simulink model "Demo_TA2_cs"  (Simulink 7.6)
settings: Solver=FixedStepDiscrete  SolverMode=SingleTasking  StartTime=0.0  StopTime=5  FixedStep=1/60  RelTol=1e-3
model workspace (MAT data in the model file):
  mbox_table.block_array(1).src = 'built-in/Subsystem'
  mbox_table.block_array(1).dest = 'Demo_TA2_cs/BMW_X5_1'
  mbox_table.block_array(1).mode = 0
  mbox_table.block_array(2).src = 'simulink/Sinks/Out1'
  mbox_table.block_array(2).dest = 'Demo_TA2_cs/BMW_X5_1/STATE_BMW_X5_1'
  mbox_table.block_array(2).mode = 0
  mbox_table.block_array(3).src = 'PreScanSimulinkLibrary/State'
  mbox_table.block_array(3).dest = 'Demo_TA2_cs/STATE_BMW_X5_1'
  mbox_table.block_array(3).mode = 0
  mbox_table.block_array(4).src = 'PreScanSimulinkLibrary/Trajectories'
  mbox_table.block_array(4).dest = 'Demo_TA2_cs/BMW_X5_1/Trajectories'
  mbox_table.block_array(4).mode = 0
  mbox_table.block_array(5).src = 'simulink/Signal Routing/Multiport Switch'
  mbox_table.block_array(5).dest = 'Demo_TA2_cs/BMW_X5_1/Trajectories/Switch'
  mbox_table.block_array(5).mode = 0
  mbox_table.block_array(6).src = 'simulink/Sources/Constant'
  mbox_table.block_array(6).dest = 'Demo_TA2_cs/BMW_X5_1/Trajectories/Trajectory_1_Offset'
  mbox_table.block_array(6).mode = 0
  mbox_table.block_array(7).src = 'PreScanSimulinkLibrary/Trajectory'
  mbox_table.block_array(7).dest = 'Demo_TA2_cs/BMW_X5_1/Trajectories/Trajectory_1'
  mbox_table.block_array(7).mode = 0
  mbox_table.block_array(8).src = 'PreScanSimulinkLibrary/Traj2State'
  mbox_table.block_array(8).dest = 'Demo_TA2_cs/BMW_X5_1/Trajectories/Traj2State1'
  mbox_table.block_array(8).mode = 0
  mbox_table.block_array(9).src = 'simulink/Sources/Constant'
  mbox_table.block_array(9).dest = 'Demo_TA2_cs/BMW_X5_1/Trajectories/Trajectory_2_Offset'
  mbox_table.block_array(9).mode = 0
  mbox_table.block_array(10).src = 'PreScanSimulinkLibrary/Trajectory'
  mbox_table.block_array(10).dest = 'Demo_TA2_cs/BMW_X5_1/Trajectories/Trajectory_2'
  mbox_table.block_array(10).mode = 0
  mbox_table.block_array(11).src = 'PreScanSimulinkLibrary/Traj2State'
  mbox_table.block_array(11).dest = 'Demo_TA2_cs/BMW_X5_1/Trajectories/Traj2State2'
  mbox_table.block_array(11).mode = 0
  mbox_table.block_array(12).src = 'simulink/Sinks/Out1'
  mbox_table.block_array(12).dest = 'Demo_TA2_cs/BMW_X5_1/Trajectories/State'
  mbox_table.block_array(12).mode = 0
  mbox_table.block_array(13).src = 'simulink/Sources/Constant'
  mbox_table.block_array(13).dest = 'Demo_TA2_cs/BMW_X5_1/Trajectories/SelectTraj'
  mbox_table.block_array(13).mode = 0
  mbox_table.block_array(14).src = 'PreScanSimulinkLibrary/SELF'
  mbox_table.block_array(14).dest = 'Demo_TA2_cs/SELF_BMW_X5_1'
  mbox_table.block_array(14).mode = 0
  mbox_table.block_array(15).src = 'simulink/Sources/In1'
  mbox_table.block_array(15).dest = 'Demo_TA2_cs/BMW_X5_1/SELF_BMW_X5_1'
  mbox_table.block_array(15).mode = 0
  mbox_table.block_array(16).src = 'PreScanSimulinkLibrary/DemuxSELF'
  mbox_table.block_array(16).dest = 'Demo_TA2_cs/BMW_X5_1/SELF_Demux'
  mbox_table.block_array(16).mode = 0
  mbox_table.block_array(17).src = 'built-in/S-Function'
  mbox_table.block_array(17).dest = 'Demo_TA2_cs/TIS_1'
  mbox_table.block_array(17).mode = 0
  mbox_table.block_array(18).src = 'simulink/Sources/In1'
  mbox_table.block_array(18).dest = 'Demo_TA2_cs/BMW_X5_1/TIS_1'
  mbox_table.block_array(18).mode = 0
  mbox_table.block_array(19).src = 'PreScanSimulinkLibrary/DemuxTIS_Standard'
  mbox_table.block_array(19).dest = 'Demo_TA2_cs/BMW_X5_1/TIS_1_Standard_Demux'
  mbox_table.block_array(19).mode = 0
  mbox_table.block_array(20).src = 'built-in/Subsystem'
  mbox_table.block_array(20).dest = 'Demo_TA2_cs/Box_1'
  mbox_table.block_array(20).mode = 0
  mbox_table.block_array(21).src = 'simulink/Sinks/Out1'
  mbox_table.block_array(21).dest = 'Demo_TA2_cs/Box_1/STATE_Box_1'
  mbox_table.block_array(21).mode = 0
  mbox_table.block_array(22).src = 'PreScanSimulinkLibrary/State'
  mbox_table.block_array(22).dest = 'Demo_TA2_cs/STATE_Box_1'
  mbox_table.block_array(22).mode = 0
  mbox_table.block_array(23).src = 'PreScanSimulinkLibrary/SELF'
  mbox_table.block_array(23).dest = 'Demo_TA2_cs/SELF_Box_1'
  mbox_table.block_array(23).mode = 0
  mbox_table.block_array(24).src = 'simulink/Sources/In1'
  mbox_table.block_array(24).dest = 'Demo_TA2_cs/Box_1/SELF_Box_1'
  mbox_table.block_array(24).mode = 0
  mbox_table.block_array(25).src = 'PreScanSimulinkLibrary/DemuxSELF'
  mbox_table.block_array(25).dest = 'Demo_TA2_cs/Box_1/SELF_Demux'
  mbox_table.block_array(25).mode = 0
  mbox_table.block_array(26).src = 'built-in/Subsystem'
  mbox_table.block_array(26).dest = 'Demo_TA2_cs/Box_1/Dynamics_Empty'
  mbox_table.block_array(26).mode = 0
  mbox_table.block_array(27).src = 'PreScanSimulinkLibrary/MuxState'
  mbox_table.block_array(27).dest = 'Demo_TA2_cs/Box_1/Dynamics_Empty/MuxState'
  mbox_table.block_array(27).mode = 0
  mbox_table.block_array(28).src = 'simulink/Sinks/Out1'
  mbox_table.block_array(28).dest = 'Demo_TA2_cs/Box_1/Dynamics_Empty/State'
  mbox_table.block_array(28).mode = 0
  mbox_table.block_array(29).src = 'built-in/Note'
  mbox_table.block_array(29).dest = 'Demo_TA2_cs/Box_1/Dynamics_Empty/For state mode ''Dynamic'' positions
    | are not taken into account, as they
    | are computed by integrating velocity.
    | Click annotation for Help.'
  mbox_table.block_array(29).mode = 0
  mbox_table.block_array(30).src = 'SimCoreLibrary/SimCoreConfiguration'
  mbox_table.block_array(30).dest = 'Demo_TA2_cs/SimCoreConfiguration'
  mbox_table.block_array(30).mode = 0
  mbox_table.block_array(31).src = 'SimCoreLibrary/Actuators'
  mbox_table.block_array(31).dest = 'Demo_TA2_cs/Actuators'
  mbox_table.block_array(31).mode = 0
  mbox_table.block_array(32).src = 'SimCoreLibrary/SetActuators'
  mbox_table.block_array(32).dest = 'Demo_TA2_cs/SetActuators'
  mbox_table.block_array(32).mode = 0
  mbox_table.block_array(33).src = 'SimCoreLibrary/GetSensors'
  mbox_table.block_array(33).dest = 'Demo_TA2_cs/GetSensors'
  mbox_table.block_array(33).mode = 0
  mbox_table.block_array(34).src = 'SimCoreLibrary/SimCoreInfo'
  mbox_table.block_array(34).dest = 'Demo_TA2_cs/SimCoreInfo'
  mbox_table.block_array(34).mode = 0
  mbox_table.block_array(35).src = 'PreScanSimulinkLibrary/Regenerate'
  mbox_table.block_array(35).dest = 'Demo_TA2_cs/Regenerate'
  mbox_table.block_array(35).mode = 0
  mbox_table.block_array(36).src = 'PreScanSimulinkLibrary/Record for Replay  '
  mbox_table.block_array(36).dest = 'Demo_TA2_cs/Record for Replay  '
  mbox_table.block_array(36).mode = 0
  mbox_table.block_array(37).src = 'PreScanSimulinkLibrary/Open Useful Blocks'
  mbox_table.block_array(37).dest = 'Demo_TA2_cs/Open Useful Blocks'
  mbox_table.block_array(37).mode = 0
  mbox_table.block_array(38).src = 'PreScanSimulinkLibrary/PreScan Options   '
  mbox_table.block_array(38).dest = 'Demo_TA2_cs/PreScan Options   '
  mbox_table.block_array(38).mode = 0
  mbox_table.block_array(39).src = 'built-in/Note'
  mbox_table.block_array(39).dest = 'Demo_TA2_cs/Version:                  '
  mbox_table.block_array(39).mode = 0
  mbox_table.block_array(40).src = 'built-in/Note'
  mbox_table.block_array(40).dest = 'Demo_TA2_cs/7.4.0'
  mbox_table.block_array(40).mode = 0
  mbox_table.block_array(41).src = 'built-in/Note'
  mbox_table.block_array(41).dest = 'Demo_TA2_cs/Author(s):                '
  mbox_table.block_array(41).mode = 0
  mbox_table.block_array(42).src = 'built-in/Note'
  mbox_table.block_array(42).dest = 'Demo_TA2_cs/D. Terra'
  mbox_table.block_array(42).mode = 0
  mbox_table.block_array(43).src = 'built-in/Note'
  mbox_table.block_array(43).dest = 'Demo_TA2_cs/Descriptive text:      '
  mbox_table.block_array(43).mode = 0
  mbox_table.block_array(44).src = 'built-in/Note'
  mbox_table.block_array(44).dest = 'Demo_TA2_cs/This experiment illustrates the
    | possibilities for Test Automation
    | that requires the PreScan
    | Experiment Editor to rebuild the
    | scenario.'
  mbox_table.block_array(44).mode = 0
  mbox_table.block_array(45).src = 'built-in/Note'
  mbox_table.block_array(45).dest = 'Demo_TA2_cs/ID
    | 
    | 4
    | 9'
  mbox_table.block_array(45).mode = 0
  mbox_table.block_array(46).src = 'built-in/Note'
  mbox_table.block_array(46).dest = 'Demo_TA2_cs/OBU-Beacon ID
    | 
    | 
    | '
  mbox_table.block_array(46).mode = 0
  mbox_table.block_array(47).src = 'built-in/Note'
  mbox_table.block_array(47).dest = 'Demo_TA2_cs/TypeID
    | 
    | 1
    | 5'
  mbox_table.block_array(47).mode = 0
  mbox_table.block_array(48).src = 'built-in/Note'
  mbox_table.block_array(48).dest = 'Demo_TA2_cs/TypeTag
    | 
    | Car
    | Cal element'
  mbox_table.block_array(48).mode = 0
  mbox_table.block_array(49).src = 'built-in/Note'
  mbox_table.block_array(49).dest = 'Demo_TA2_cs/SD
    | 
    | Y
    | Y'
  mbox_table.block_array(49).mode = 0
  mbox_table.block_array(50).src = 'built-in/Note'
  mbox_table.block_array(50).dest = 'Demo_TA2_cs/CD
    | 
    | N
    | N'
  mbox_table.block_array(50).mode = 0
  mbox_table.block_array(51).src = 'built-in/Note'
  mbox_table.block_array(51).dest = 'Demo_TA2_cs/Name
    | 
    | BMW_X5_1
    | Box_1'
  mbox_table.block_array(51).mode = 0
  mbox_table.block_array(52).src = 'built-in/Note'
  mbox_table.block_array(52).dest = 'Demo_TA2_cs/Num ID       OBU-Beacon ID     Type ID      Type Tag             SD        CD             Name                          '
  mbox_table.block_array(52).mode = 0
  mbox_table.block_array(53).src = 'built-in/Terminator'
  mbox_table.block_array(53).dest = 'Demo_TA2_cs/BMW_X5_1/Terminator_1'
  mbox_table.block_array(53).mode = 1
  mbox_table.block_array(54).src = 'built-in/Terminator'
  mbox_table.block_array(54).dest = 'Demo_TA2_cs/BMW_X5_1/Terminator_2'
  mbox_table.block_array(54).mode = 1
  mbox_table.block_array(55).src = 'built-in/Terminator'
  mbox_table.block_array(55).dest = 'Demo_TA2_cs/BMW_X5_1/Terminator_3'
  mbox_table.block_array(55).mode = 1
  mbox_table.block_array(56).src = 'built-in/Terminator'
  mbox_table.block_array(56).dest = 'Demo_TA2_cs/BMW_X5_1/Terminator_4'
  mbox_table.block_array(56).mode = 1
  mbox_table.block_array(57).src = 'built-in/Terminator'
  mbox_table.block_array(57).dest = 'Demo_TA2_cs/BMW_X5_1/Terminator_5'
  mbox_table.block_array(57).mode = 1
  mbox_table.block_array(58).src = 'built-in/Terminator'
  mbox_table.block_array(58).dest = 'Demo_TA2_cs/BMW_X5_1/Terminator_6'
  mbox_table.block_array(58).mode = 1
  mbox_table.block_array(59).src = 'built-in/Terminator'
  mbox_table.block_array(59).dest = 'Demo_TA2_cs/BMW_X5_1/Terminator_7'
  mbox_table.block_array(59).mode = 1
  mbox_table.block_array(60).src = 'built-in/Terminator'
  mbox_table.block_array(60).dest = 'Demo_TA2_cs/BMW_X5_1/Terminator_8'
  mbox_table.block_array(60).mode = 1
  mbox_table.block_array(61).src = 'built-in/Terminator'
  mbox_table.block_array(61).dest = 'Demo_TA2_cs/BMW_X5_1/Terminator_9'
  mbox_table.block_array(61).mode = 1
  mbox_table.block_array(62).src = 'built-in/Terminator'
  mbox_table.block_array(62).dest = 'Demo_TA2_cs/BMW_X5_1/Terminator_10'
  mbox_table.block_array(62).mode = 1
  mbox_table.block_array(63).src = 'built-in/Terminator'
  mbox_table.block_array(63).dest = 'Demo_TA2_cs/BMW_X5_1/Terminator_11'
  mbox_table.block_array(63).mode = 1
  mbox_table.block_array(64).src = 'built-in/Terminator'
  mbox_table.block_array(64).dest = 'Demo_TA2_cs/BMW_X5_1/Terminator_12'
  mbox_table.block_array(64).mode = 1
  mbox_table.block_array(65).src = 'built-in/Terminator'
  mbox_table.block_array(65).dest = 'Demo_TA2_cs/BMW_X5_1/Terminator_13'
  mbox_table.block_array(65).mode = 1
  mbox_table.block_array(66).src = 'built-in/Terminator'
  mbox_table.block_array(66).dest = 'Demo_TA2_cs/BMW_X5_1/Terminator_14'
  mbox_table.block_array(66).mode = 1
  mbox_table.block_array(67).src = 'built-in/Terminator'
  mbox_table.block_array(67).dest = 'Demo_TA2_cs/BMW_X5_1/Terminator_15'
  mbox_table.block_array(67).mode = 1
  mbox_table.block_array(68).src = 'built-in/Terminator'
  mbox_table.block_array(68).dest = 'Demo_TA2_cs/BMW_X5_1/Terminator_16'
  mbox_table.block_array(68).mode = 1
  mbox_table.block_index : java.util.Hashtable (value not decoded)
  mbox_table.line_array(1).sys = 'Demo_TA2_cs'
  mbox_table.line_array(1).line_id = 'L1'
  mbox_table.line_array(1).iport = 'STATE_BMW_X5_1/1'
  mbox_table.line_array(1).oport = 'BMW_X5_1/1'
  mbox_table.line_array(1).mode = 0
  mbox_table.line_array(2).sys = 'Demo_TA2_cs/BMW_X5_1/Trajectories'
  mbox_table.line_array(2).line_id = 'L2'
  mbox_table.line_array(2).iport = 'Traj2State1/1'
  mbox_table.line_array(2).oport = 'Trajectory_1/1'
  mbox_table.line_array(2).mode = 0
  mbox_table.line_array(3).sys = 'Demo_TA2_cs/BMW_X5_1/Trajectories'
  mbox_table.line_array(3).line_id = 'L3'
  mbox_table.line_array(3).iport = 'Traj2State1/2'
  mbox_table.line_array(3).oport = 'Trajectory_1_Offset/1'
  mbox_table.line_array(3).mode = 0
  mbox_table.line_array(4).sys = 'Demo_TA2_cs/BMW_X5_1/Trajectories'
  mbox_table.line_array(4).line_id = 'L4'
  mbox_table.line_array(4).iport = 'Switch/2'
  mbox_table.line_array(4).oport = 'Traj2State1/1'
  mbox_table.line_array(4).mode = 0
  mbox_table.line_array(5).sys = 'Demo_TA2_cs/BMW_X5_1/Trajectories'
  mbox_table.line_array(5).line_id = 'L5'
  mbox_table.line_array(5).iport = 'Traj2State2/1'
  mbox_table.line_array(5).oport = 'Trajectory_2/1'
  mbox_table.line_array(5).mode = 0
  mbox_table.line_array(6).sys = 'Demo_TA2_cs/BMW_X5_1/Trajectories'
  mbox_table.line_array(6).line_id = 'L6'
  mbox_table.line_array(6).iport = 'Traj2State2/2'
  mbox_table.line_array(6).oport = 'Trajectory_2_Offset/1'
  mbox_table.line_array(6).mode = 0
  mbox_table.line_array(7).sys = 'Demo_TA2_cs/BMW_X5_1/Trajectories'
  mbox_table.line_array(7).line_id = 'L7'
  mbox_table.line_array(7).iport = 'Switch/3'
  mbox_table.line_array(7).oport = 'Traj2State2/1'
  mbox_table.line_array(7).mode = 0
  mbox_table.line_array(8).sys = 'Demo_TA2_cs/BMW_X5_1/Trajectories'
  mbox_table.line_array(8).line_id = 'L8'
  mbox_table.line_array(8).iport = 'Switch/1'
  mbox_table.line_array(8).oport = 'SelectTraj/1'
  mbox_table.line_array(8).mode = 0
  mbox_table.line_array(9).sys = 'Demo_TA2_cs/BMW_X5_1/Trajectories'
  mbox_table.line_array(9).line_id = 'L9'
  mbox_table.line_array(9).iport = 'State/1'
  mbox_table.line_array(9).oport = 'Switch/1'
  mbox_table.line_array(9).mode = 0
  mbox_table.line_array(10).sys = 'Demo_TA2_cs'
  mbox_table.line_array(10).line_id = 'L10'
  mbox_table.line_array(10).iport = 'BMW_X5_1/1'
  mbox_table.line_array(10).oport = 'SELF_BMW_X5_1/1'
  mbox_table.line_array(10).mode = 0
  mbox_table.line_array(11).sys = 'Demo_TA2_cs/BMW_X5_1'
  mbox_table.line_array(11).line_id = 'L11'
  mbox_table.line_array(11).iport = 'SELF_Demux/1'
  mbox_table.line_array(11).oport = 'SELF_BMW_X5_1/1'
  mbox_table.line_array(11).mode = 0
  mbox_table.line_array(12).sys = 'Demo_TA2_cs'
  mbox_table.line_array(12).line_id = 'L12'
  mbox_table.line_array(12).iport = 'BMW_X5_1/2'
  mbox_table.line_array(12).oport = 'TIS_1/1'
  mbox_table.line_array(12).mode = 0
  mbox_table.line_array(13).sys = 'Demo_TA2_cs/BMW_X5_1'
  mbox_table.line_array(13).line_id = 'L13'
  mbox_table.line_array(13).iport = 'TIS_1_Standard_Demux/1'
  mbox_table.line_array(13).oport = 'TIS_1/1'
  mbox_table.line_array(13).mode = 0
  mbox_table.line_array(14).sys = 'Demo_TA2_cs/BMW_X5_1'
  mbox_table.line_array(14).line_id = 'L14'
  mbox_table.line_array(14).iport = 'STATE_BMW_X5_1/1'
  mbox_table.line_array(14).oport = 'Trajectories/1'
  mbox_table.line_array(14).mode = 0
  mbox_table.line_array(15).sys = 'Demo_TA2_cs'
  mbox_table.line_array(15).line_id = 'L15'
  mbox_table.line_array(15).iport = 'STATE_Box_1/1'
  mbox_table.line_array(15).oport = 'Box_1/1'
  mbox_table.line_array(15).mode = 0
  mbox_table.line_array(16).sys = 'Demo_TA2_cs'
  mbox_table.line_array(16).line_id = 'L16'
  mbox_table.line_array(16).iport = 'Box_1/1'
  mbox_table.line_array(16).oport = 'SELF_Box_1/1'
  mbox_table.line_array(16).mode = 0
  mbox_table.line_array(17).sys = 'Demo_TA2_cs/Box_1'
  mbox_table.line_array(17).line_id = 'L17'
  mbox_table.line_array(17).iport = 'SELF_Demux/1'
  mbox_table.line_array(17).oport = 'SELF_Box_1/1'
  mbox_table.line_array(17).mode = 0
  mbox_table.line_array(18).sys = 'Demo_TA2_cs/Box_1/Dynamics_Empty'
  mbox_table.line_array(18).line_id = 'L18'
  mbox_table.line_array(18).iport = 'State/1'
  mbox_table.line_array(18).oport = 'MuxState/1'
  mbox_table.line_array(18).mode = 0
  mbox_table.line_array(19).sys = 'Demo_TA2_cs/Box_1'
  mbox_table.line_array(19).line_id = 'L19'
  mbox_table.line_array(19).iport = 'STATE_Box_1/1'
  mbox_table.line_array(19).oport = 'Dynamics_Empty/1'
  mbox_table.line_array(19).mode = 0
  mbox_table.line_array(20).sys = 'Demo_TA2_cs/BMW_X5_1'
  mbox_table.line_array(20).line_id = 'l1'
  mbox_table.line_array(20).iport = 'Terminator_1/1'
  mbox_table.line_array(20).oport = 'SELF_Demux/1'
  mbox_table.line_array(20).mode = 1
  mbox_table.line_array(21).sys = 'Demo_TA2_cs/BMW_X5_1'
  mbox_table.line_array(21).line_id = 'l2'
  mbox_table.line_array(21).iport = 'Terminator_2/1'
  mbox_table.line_array(21).oport = 'SELF_Demux/2'
  mbox_table.line_array(21).mode = 1
  mbox_table.line_array(22).sys = 'Demo_TA2_cs/BMW_X5_1'
  mbox_table.line_array(22).line_id = 'l3'
  mbox_table.line_array(22).iport = 'Terminator_3/1'
  mbox_table.line_array(22).oport = 'SELF_Demux/3'
  mbox_table.line_array(22).mode = 1
  mbox_table.line_array(23).sys = 'Demo_TA2_cs/BMW_X5_1'
  mbox_table.line_array(23).line_id = 'l4'
  mbox_table.line_array(23).iport = 'Terminator_4/1'
  mbox_table.line_array(23).oport = 'SELF_Demux/4'
  mbox_table.line_array(23).mode = 1
  mbox_table.line_array(24).sys = 'Demo_TA2_cs/BMW_X5_1'
  mbox_table.line_array(24).line_id = 'l5'
  mbox_table.line_array(24).iport = 'Terminator_5/1'
  mbox_table.line_array(24).oport = 'SELF_Demux/5'
  mbox_table.line_array(24).mode = 1
  mbox_table.line_array(25).sys = 'Demo_TA2_cs/BMW_X5_1'
  mbox_table.line_array(25).line_id = 'l6'
  mbox_table.line_array(25).iport = 'Terminator_6/1'
  mbox_table.line_array(25).oport = 'SELF_Demux/6'
  mbox_table.line_array(25).mode = 1
  mbox_table.line_array(26).sys = 'Demo_TA2_cs/BMW_X5_1'
  mbox_table.line_array(26).line_id = 'l7'
  mbox_table.line_array(26).iport = 'Terminator_7/1'
  mbox_table.line_array(26).oport = 'SELF_Demux/7'
  mbox_table.line_array(26).mode = 1
  mbox_table.line_array(27).sys = 'Demo_TA2_cs/BMW_X5_1'
  mbox_table.line_array(27).line_id = 'l8'
  mbox_table.line_array(27).iport = 'Terminator_8/1'
  mbox_table.line_array(27).oport = 'SELF_Demux/8'
  mbox_table.line_array(27).mode = 1
  mbox_table.line_array(28).sys = 'Demo_TA2_cs/BMW_X5_1'
  mbox_table.line_array(28).line_id = 'l9'
  mbox_table.line_array(28).iport = 'Terminator_9/1'
  mbox_table.line_array(28).oport = 'SELF_Demux/9'
  mbox_table.line_array(28).mode = 1
  mbox_table.line_array(29).sys = 'Demo_TA2_cs/BMW_X5_1'
  mbox_table.line_array(29).line_id = 'l10'
  mbox_table.line_array(29).iport = 'Terminator_10/1'
  mbox_table.line_array(29).oport = 'SELF_Demux/10'
  mbox_table.line_array(29).mode = 1
  mbox_table.line_array(30).sys = 'Demo_TA2_cs/BMW_X5_1'
  mbox_table.line_array(30).line_id = 'l11'
  mbox_table.line_array(30).iport = 'Terminator_11/1'
  mbox_table.line_array(30).oport = 'SELF_Demux/11'
  mbox_table.line_array(30).mode = 1
  mbox_table.line_array(31).sys = 'Demo_TA2_cs/BMW_X5_1'
  mbox_table.line_array(31).line_id = 'l12'
  mbox_table.line_array(31).iport = 'Terminator_12/1'
  mbox_table.line_array(31).oport = 'SELF_Demux/12'
  mbox_table.line_array(31).mode = 1
  mbox_table.line_array(32).sys = 'Demo_TA2_cs/BMW_X5_1'
  mbox_table.line_array(32).line_id = 'l13'
  mbox_table.line_array(32).iport = 'Terminator_13/1'
  mbox_table.line_array(32).oport = 'TIS_1_Standard_Demux/3'
  mbox_table.line_array(32).mode = 1
  mbox_table.line_array(33).sys = 'Demo_TA2_cs/BMW_X5_1'
  mbox_table.line_array(33).line_id = 'l14'
  mbox_table.line_array(33).iport = 'Terminator_14/1'
  mbox_table.line_array(33).oport = 'TIS_1_Standard_Demux/4'
  mbox_table.line_array(33).mode = 1
  mbox_table.line_array(34).sys = 'Demo_TA2_cs/BMW_X5_1'
  mbox_table.line_array(34).line_id = 'l15'
  mbox_table.line_array(34).iport = 'Terminator_15/1'
  mbox_table.line_array(34).oport = 'TIS_1_Standard_Demux/5'
  mbox_table.line_array(34).mode = 1
  mbox_table.line_array(35).sys = 'Demo_TA2_cs/BMW_X5_1'
  mbox_table.line_array(35).line_id = 'l16'
  mbox_table.line_array(35).iport = 'Terminator_16/1'
  mbox_table.line_array(35).oport = 'TIS_1_Standard_Demux/6'
  mbox_table.line_array(35).mode = 1
  mbox_table.line_index : java.util.Hashtable (value not decoded)
  mbox_table.next_linenr = 20
  mbox_table.next_termlinenr = 17
  model_closed = 0
  sim_status = 0
PreLoadFcn:
  | check_NUTS_defined;
  | 
  | assignin('base',['model_closed_' bdroot],false);
InitFcn:
  | PreScanExperimentInitFcn(bdroot)
StopFcn:
  | PreScanExperimentStopFcn(bdroot)
undefined symbols (not defined in the file or in its folder): DiscIntNeverNeededParam
libraries: PreScanSimulinkLibrary x9, PreScanUsefulBlocks x3
(part 1 of 2)
CloseFcn:
  | evalin('base',['clear model_closed_' bdroot]);
settings Model: Creator=PRESCAN  LastModifiedBy=buildbot
settings OptimizationCC: InitFltsAndDblsToZero=on
settings DebuggingCC: SaveWithParameterizedLinksMsg=none  SignalResolutionControl=TryResolveAllWithWarning  MultiTaskDSMMsg=warning  MultiTaskCondExecSysMsg=none
settings RTWCC: IncludeERTFirstTime=on
settings GRTTargetCC: TargetFcnLib=ansi_tfl_tmw.mat

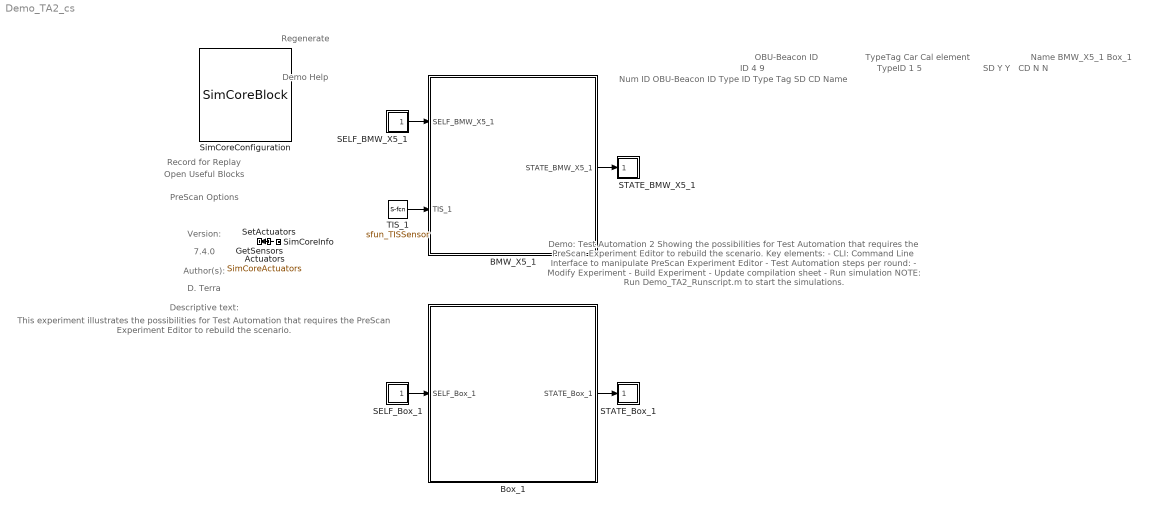
== system Demo_TA2_cs ==
  note: Demo: Test Automation 2
      | Showing the possibilities for Test Automation that requires the PreScan
      | Experiment Editor to rebuild the scenario.
      |
      | Key elements:
      | - CLI: Command Line Interface to manipulate PreScan Experiment Editor
      | - Test Automation steps per round:
      |     - Modify Experiment
      |     - Build Experiment
      |     - Update compilation sheet
      |     - Run simulation
      |
      | NOTE:
      | Run Demo_TA2_Runscript.m to start the simulations.
  note: Demo Help
  note: Regenerate
  note: Record for Replay
  note: Open Useful Blocks
  note: PreScan Options
  note: Version:
  note: 7.4.0
  note: Author(s):
  note: D. Terra
  note: Descriptive text:
  note: This experiment illustrates the
      | possibilities for Test Automation
      | that requires the PreScan
      | Experiment Editor to rebuild the
      | scenario.
  note: ID
      |
      | 4
      | 9
  note: OBU-Beacon ID
  note: TypeID
      |
      | 1
      | 5
  note: TypeTag
      |
      | Car
      | Cal element
  note: SD
      |
      | Y
      | Y
  note: CD
      |
      | N
      | N
  note: Name
      |
      | BMW_X5_1
      | Box_1
  note: Num ID OBU-Beacon ID Type ID Type Tag SD CD Name
  Actuators : DataStoreMemory  Tag=Actuators  DataStoreName=SimCoreActuators  InitialValue=zeros(30,1)
      settings: DeleteFcn=PreScanBlockDeleteFcn;
  BMW_X5_1 : Subsystem  Tag=WorldObjectSubSystem  InitFcn=UniqueId = '33';
      mask Display: image(imread('BMW_X5.jpg'));color('white');text(0,0,' ID=4\n')
  Box_1 : Subsystem  Tag=WorldObjectSubSystem  InitFcn=UniqueId = '41';
      mask Display: image(imread('Box.jpg'));color('white');text(0,0,' ID=9\n')
  GetSensors : Subsystem  Tag=GetSensors  Priority=2  mask(PreScan Simulation Core Block){NrOfSensors=16, TimeStep=1/60}
      mask prompts: NrOfSensors "Number of sensor values"; TimeStep "Timestep [s]"
      mask help:
      | Please do not remove this block from the PreScan compilation sheet,
      | as it contains essential configuration parameters for a PreScan simulation.
      settings: DeleteFcn=PreScanBlockDeleteFcn;
  SELF_BMW_X5_1 : Subsystem  Tag=SELF  Priority=3  mask(PreScan Source Block: SELF){PortName=SELF_BMW_X5_1, PortIndex=0, PortWidth=8, TimeStep=1/60}
      mask prompts: PortName "Auto-Assigned: Port Name [-]"; PortIndex "Auto-Assigned: Port Index [-]"; PortWidth "Auto-Assigned: Port Dimensions"; TimeStep "Auto-Assigned: Upload Period [s]"
      mask help:
      | The SELF port shows (state) information of the actor itself. The outputs are position in the experiment's axis system and the GPS coordinates, and the object's absolute velocity and compass heading.
      |
      | For more information, please click Help.
      settings: DeleteFcn=PreScanBlockDeleteFcn;
      mask Help: eval('openHelp(462)')
      mask Display: image(imread('GPS.png'))
  SELF_Box_1 : Subsystem  Tag=SELF  Priority=3  mask(PreScan Source Block: SELF){PortName=SELF_Box_1, PortIndex=8, PortWidth=8, TimeStep=1/60}
      mask prompts: PortName "Auto-Assigned: Port Name [-]"; PortIndex "Auto-Assigned: Port Index [-]"; PortWidth "Auto-Assigned: Port Dimensions"; TimeStep "Auto-Assigned: Upload Period [s]"
      mask help:
      | The SELF port shows (state) information of the actor itself. The outputs are position in the experiment's axis system and the GPS coordinates, and the object's absolute velocity and compass heading.
      |
      | For more information, please click Help.
      settings: DeleteFcn=PreScanBlockDeleteFcn;
      mask Help: eval('openHelp(462)')
      mask Display: image(imread('GPS.png'))
  STATE_BMW_X5_1 : Subsystem  Tag=State  Priority=0  mask(PreScan Sink Block: State){x0=0, y0=-1.75, z0=0.68999999761581421, Roll0=0, Pitch0=0, Yaw0=0, TimeStep=1/60}
      mask prompts: x0 "Ini x-position VEHICLE wrt GLOBAL axis system [m]"; y0 "Ini y-position VEHICLE wrt GLOBAL axis system [m]"; z0 "Ini z-position VEHICLE wrt GLOBAL axis system [m]"; Roll0 "Ini roll-angle BODY wrt VEHICLE axis system [deg]"; Pitch0 "Ini pitch-angle BODY wrt VEHICLE axis system [deg]"; Yaw0 "Ini yaw-angle VEHICLE wrt GLOBAL axis system [deg]"; TimeStep "Time Step [s]"
      mask help:
      | The Actor State contains a vector signal of size (9x1), containing the following signals:
      |
      | -  Position                  (x,y,z)                                     [m]
      | -  Velocity                  (vx,vy,vz)                               [m/s]
      | -  Angles                    (Roll, Pitch, Yaw)                   [rad]
      |
      | The Actor state is defined in the global axis system.
      | The state is superponed on the Initial position defined in the GUI.
      |
      | For more information, please click Help.
      settings: DeleteFcn=PreScanBlockDeleteFcn;
      mask Help: eval('openHelp(222)')
      mask Display: image(imread('State.png'))
  STATE_Box_1 : Subsystem  Tag=State  Priority=0  mask(PreScan Sink Block: State){x0=38, y0=0, z0=0, Roll0=0, Pitch0=0, Yaw0=0, TimeStep=1/60}
      mask prompts: x0 "Ini x-position VEHICLE wrt GLOBAL axis system [m]"; y0 "Ini y-position VEHICLE wrt GLOBAL axis system [m]"; z0 "Ini z-position VEHICLE wrt GLOBAL axis system [m]"; Roll0 "Ini roll-angle BODY wrt VEHICLE axis system [deg]"; Pitch0 "Ini pitch-angle BODY wrt VEHICLE axis system [deg]"; Yaw0 "Ini yaw-angle VEHICLE wrt GLOBAL axis system [deg]"; TimeStep "Time Step [s]"
      mask help:
      | The Actor State contains a vector signal of size (9x1), containing the following signals:
      |
      | -  Position                  (x,y,z)                                     [m]
      | -  Velocity                  (vx,vy,vz)                               [m/s]
      | -  Angles                    (Roll, Pitch, Yaw)                   [rad]
      |
      | The Actor state is defined in the global axis system.
      | The state is superponed on the Initial position defined in the GUI.
      |
      | For more information, please click Help.
      settings: DeleteFcn=PreScanBlockDeleteFcn;
      mask Help: eval('openHelp(222)')
      mask Display: image(imread('State.png'))
  SetActuators : Subsystem  Tag=SetActuators  Priority=1  mask(PreScan Simulation Core Block){TimeStep=1/60, NrOfActuators=30}
      mask prompts: TimeStep "Timestep [s]"; NrOfActuators "Number of actuator values"
      mask help:
      | Please do not remove this block from the PreScan compilation sheet,
      | as it contains essential configuration parameters for a PreScan simulation.
      settings: DeleteFcn=PreScanBlockDeleteFcn;
  SimCoreConfiguration : M-S-Function  Tag=SimCoreConfiguration  Description=839168CDEDD100B1BE966240BE789E2F4508DB343ED6100BC12AAB51D6F7B04F  FunctionName=SimCoreBlock  Parameters=ExperimentXML PortsXML SimulationCore HostName CheckStart EnableLog RfR EnableGPUAccel ShowComputationTime  mask(PreScan Simulation Core Configurator){SimulationCore=NUTS, HostName=0, CheckStart=0, prescanversion='7.4.0', EnableLog=off, RfR=0, EnableGPUAccel=off, ShowComputationTime=off}
      mask prompts: SimulationCore "Simulation Core"; HostName "Simulation Host"; CheckStart "Show START Dialog"; prescanversion "PreScan Version"; EnableLog "Create TA Log"; RfR "Record for Replay"; EnableGPUAccel "Enable GPU Acceleration"; ShowComputationTime "Show ComputationTime Scope"
      mask help:
      | Please do not remove this block from the PreScan compilation sheet,
      | as it contains essential configuration parameter for a PreScan simulation.
      mask init:
      | model = bdroot;
      | ExperimentXML = [model(1:end-3) '.pex'];
      | PortsXML = [model '_ports.pcd'];
      settings: DeleteFcn=PreScanBlockDeleteFcn;  ModelCloseFcn=assignin('base',['model_closed_' bdroot],true);
      mask Help: eval('openHelp(812)')
      mask Display: image(imread('prescanlogo.ico'))
  SimCoreInfo : Subsystem  Tag=SimCoreInfo
  TIS_1 : S-Function  Priority=3  LoadFcn=load('PrescanScannerSensorData.mat');load('PrescanScannerSensorMessage.mat')  FunctionName=sfun_TISSensor  Parameters=timestepMask maxInputMessages maxOutputMessages sensorID detectableObjects  EnableBusSupport=off  mask{timestepMask=1/60, maxInputMessages=0, maxOutputMessages=1, sensorID=40, detectableObjects=1}
      mask prompts: timestepMask "MATLAB timestep:"; maxInputMessages "Max input messages:"; maxOutputMessages "Max output messages:"; sensorID "Sensor ID:"; detectableObjects "Max detectable objects:"
      mask help: TIS Sensor I/O
      mask Display: image(imread('TIS.png'))
  wires:
  BMW_X5_1/1(STATE_BMW_X5_1) -> STATE_BMW_X5_1/1(State)
  SELF_BMW_X5_1/1(U) -> BMW_X5_1/1(SELF_BMW_X5_1)
  TIS_1/1 -> BMW_X5_1/2(TIS_1)
  Box_1/1(STATE_Box_1) -> STATE_Box_1/1(State)
  SELF_Box_1/1(U) -> Box_1/1(SELF_Box_1)
  SetActuators/1(dummy) -> GetSensors/1(dummy)

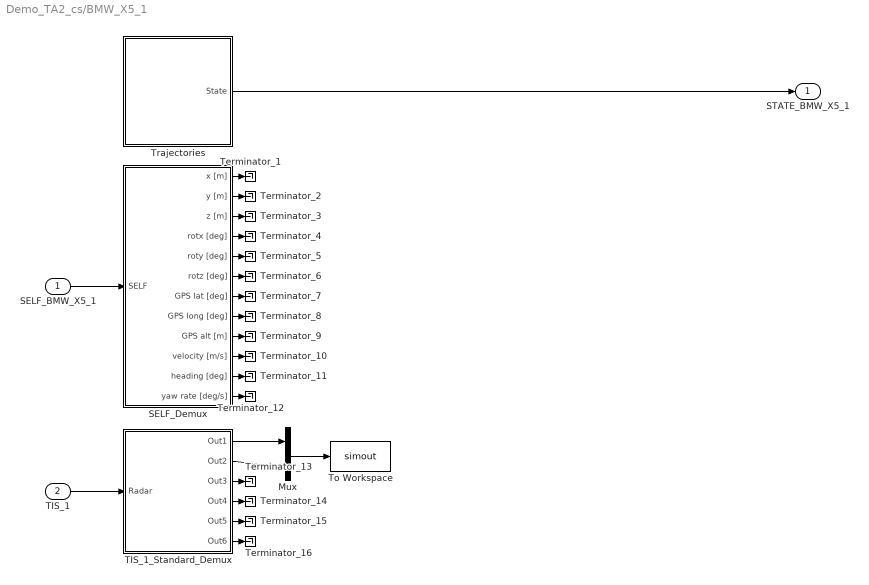
== system Demo_TA2_cs/BMW_X5_1 ==
  SELF_BMW_X5_1 : Inport  Tag=SELFInport
  TIS_1 : Inport  Tag=RadarInport  Port=2  OutDataTypeStr=Bus: PRESCAN_SCANNERSENSORMESSAGE
  Mux : Mux  Inputs=2
  SELF_Demux : Subsystem  Tag=DemuxSELF
      settings: DeleteFcn=PreScanBlockDeleteFcn;
      mask Type: PreScan Demux Block:
      mask Display:
      | port_label('output',1,'x [m]')
      | port_label('output',2,'y [m]')
      | port_label('output',3,'z [m]','texmode','on')
      | port_label('output',4,'Rotx [deg]','texmode','on')
      | port_label('output',5,'Roty [deg]','texmode','on')
      | port_label('output',6,'Rotz [deg]','texmode','on')
      | port_label('output',7,'GPS lat [deg]','texmode','on')
      | port_label('output',8,'GPS long [deg]','texmode','on')
      | port_label('output',9,'GPS alt [m]','texmode','on')
      | port_label('output',10,'Velocity [m/s]')
      | port_label('output',11,'Heading [deg]')
      | port_label('output',12,'Yaw rate [deg/s]')
  TIS_1_Standard_Demux : Subsystem  TreatAsAtomicUnit=on  mask(PreScan Demux Block: TIS){MAXMESSAGES=1}
      mask prompts: MAXMESSAGES "Number of Objects"
      mask Help: eval('openHelp(441)')
      mask Display:
      | port_label('input',1,'TIS')
      | port_label('output',1,'Beam ID [-]')
      | port_label('output',2,'Range [m]')
      | port_label('output',3,'{\theta} [deg]','texmode','on')
      | port_label('output',4,'{\phi} [deg]','texmode','on')
      | port_label('output',5,'Target ID [-]','texmode','on')
      | port_label('output',6,'TIS Data','texmode','on')
  Terminator_{1..16} (16 alike) : Terminator
  To Workspace : ToWorkspace  VariableName=simout  SampleTime=-1  SaveFormat=Array
  Trajectories : Subsystem  Tag=Trajectories
      settings: DeleteFcn=PreScanBlockDeleteFcn;
      mask Display: image(imread('Trajectory.png'));
  STATE_BMW_X5_1 : Outport  Tag=StateOutport
  wires:
  Mux/1 -> To Workspace/1
  SELF_BMW_X5_1/1 -> SELF_Demux/1(SELF)
  TIS_1/1 -> TIS_1_Standard_Demux/1(Radar)
  Trajectories/1(State) -> STATE_BMW_X5_1/1
  TIS_1_Standard_Demux/1(Out1) -> Mux/1
  TIS_1_Standard_Demux/2(Out2) -> Mux/2
  SELF_Demux/1(x [m]) -> Terminator_1/1
  SELF_Demux/2(y [m]) -> Terminator_2/1
  SELF_Demux/3(z [m]) -> Terminator_3/1
  SELF_Demux/4(rotx [deg]) -> Terminator_4/1
  SELF_Demux/5(roty [deg]) -> Terminator_5/1
  SELF_Demux/6(rotz [deg]) -> Terminator_6/1
  SELF_Demux/7(GPS lat [deg]) -> Terminator_7/1
  SELF_Demux/8(GPS long [deg]) -> Terminator_8/1
  SELF_Demux/9(GPS alt [m]) -> Terminator_9/1
  SELF_Demux/10(velocity [m/s]) -> Terminator_10/1
  SELF_Demux/11(heading [deg]) -> Terminator_11/1
  SELF_Demux/12(yaw rate [deg/s]) -> Terminator_12/1
  TIS_1_Standard_Demux/3(Out3) -> Terminator_13/1
  TIS_1_Standard_Demux/4(Out4) -> Terminator_14/1
  TIS_1_Standard_Demux/5(Out5) -> Terminator_15/1
  TIS_1_Standard_Demux/6(Out6) -> Terminator_16/1

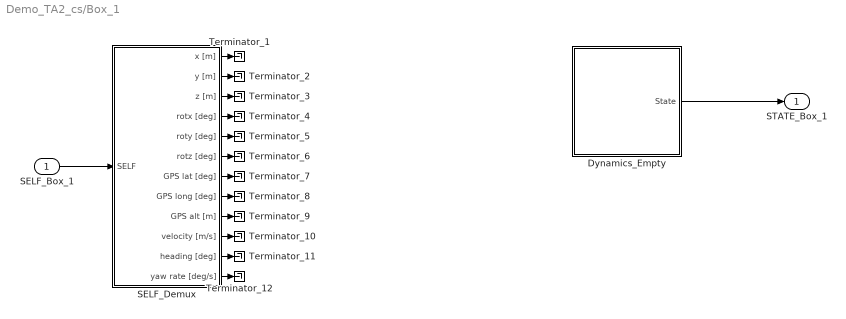
== system Demo_TA2_cs/Box_1 ==
  SELF_Box_1 : Inport  Tag=SELFInport
  Dynamics_Empty : Subsystem  Tag=Dynamics_Empty
      mask Display: port_label('output', 1, 'State');text(0,0,' Empty\n')
  SELF_Demux : Subsystem  Tag=DemuxSELF
      settings: DeleteFcn=PreScanBlockDeleteFcn;
      mask Type: PreScan Demux Block:
      mask Display:
      | port_label('output',1,'x [m]')
      | port_label('output',2,'y [m]')
      | port_label('output',3,'z [m]','texmode','on')
      | port_label('output',4,'Rotx [deg]','texmode','on')
      | port_label('output',5,'Roty [deg]','texmode','on')
      | port_label('output',6,'Rotz [deg]','texmode','on')
      | port_label('output',7,'GPS lat [deg]','texmode','on')
      | port_label('output',8,'GPS long [deg]','texmode','on')
      | port_label('output',9,'GPS alt [m]','texmode','on')
      | port_label('output',10,'Velocity [m/s]')
      | port_label('output',11,'Heading [deg]')
      | port_label('output',12,'Yaw rate [deg/s]')
  Terminator_{1..12} (12 alike) : Terminator
  STATE_Box_1 : Outport  Tag=StateOutport
  wires:
  SELF_Box_1/1 -> SELF_Demux/1(SELF)
  Dynamics_Empty/1(State) -> STATE_Box_1/1
  SELF_Demux/1(x [m]) -> Terminator_1/1
  SELF_Demux/2(y [m]) -> Terminator_2/1
  SELF_Demux/3(z [m]) -> Terminator_3/1
  SELF_Demux/4(rotx [deg]) -> Terminator_4/1
  SELF_Demux/5(roty [deg]) -> Terminator_5/1
  SELF_Demux/6(rotz [deg]) -> Terminator_6/1
  SELF_Demux/7(GPS lat [deg]) -> Terminator_7/1
  SELF_Demux/8(GPS long [deg]) -> Terminator_8/1
  SELF_Demux/9(GPS alt [m]) -> Terminator_9/1
  SELF_Demux/10(velocity [m/s]) -> Terminator_10/1
  SELF_Demux/11(heading [deg]) -> Terminator_11/1
  SELF_Demux/12(yaw rate [deg/s]) -> Terminator_12/1

== system Demo_TA2_cs/GetSensors ==
  dummy : Inport
  GetSensors : M-S-Function  FunctionName=GetSensorsBlock  Parameters=TimeStep NrOfSensors
  tag scope: SimCoreSensors=global
  wires:
  GetSensors/1 -> [SimCoreSensors]
  dummy/1 -> GetSensors/1

== system Demo_TA2_cs/SELF_BMW_X5_1 ==
  Selector : Selector  IndexMode=Zero-based  IndexOptions=Starting index (dialog)  Indices=PortIndex  OutputSizes=PortWidth(1)
  U : Outport
  wires:
  Selector/1 -> U/1
  [SimCoreSensors] -> Selector/1

== system Demo_TA2_cs/SELF_Box_1 ==
  Selector : Selector  IndexMode=Zero-based  IndexOptions=Starting index (dialog)  Indices=PortIndex  OutputSizes=PortWidth(1)
  U : Outport
  wires:
  Selector/1 -> U/1
  [SimCoreSensors] -> Selector/1

== system Demo_TA2_cs/STATE_BMW_X5_1 ==
  State : Inport  SampleTime=TimeStep
  Acceleration : Subsystem  mask(ToSensorWorld){PortName=Acceleration_BMW_X5_1, PortIndex=6, PortWidth=3, TimeStep=1/60}
      mask prompts: PortName "Port Name [-]"; PortIndex "Index [-]"; PortWidth "Port Dimensions [-]"; TimeStep "Upload Period [s]"
      mask help: Sends signal(s) from Simulink to the Sensor World
      mask Help:
      | Sends signal(s) from Simulink to the Sensor World.
      | 
      | - Port Name [-]: specifies the name of the output terminal of the Simulink block.
      | - Index [-]: specifies the start position in the output vector sent to the Sensor World
      | - Port dimensions [-]: specifies the width (number of scalars) of the output port
      | - Upload period [s]: specifies the upload period (in seconds) of the port.
      mask Display: port_label('input', 1, PortName)
  Demux : Demux  Outputs=5
  Position : Subsystem  mask(ToSensorWorld){PortName=Position_BMW_X5_1, PortIndex=0, PortWidth=3, TimeStep=1/60}
      mask prompts: PortName "Port Name [-]"; PortIndex "Index [-]"; PortWidth "Port Dimensions [-]"; TimeStep "Upload Period [s]"
      mask help: Sends signal(s) from Simulink to the Sensor World
      mask Help:
      | Sends signal(s) from Simulink to the Sensor World.
      | 
      | - Port Name [-]: specifies the name of the output terminal of the Simulink block.
      | - Index [-]: specifies the start position in the output vector sent to the Sensor World
      | - Port dimensions [-]: specifies the width (number of scalars) of the output port
      | - Upload period [s]: specifies the upload period (in seconds) of the port.
      mask Display: port_label('input', 1, PortName)
  RPY : Subsystem  mask(ToSensorWorld){PortName=RPY_BMW_X5_1, PortIndex=9, PortWidth=3, TimeStep=1/60}
      mask prompts: PortName "Port Name [-]"; PortIndex "Index [-]"; PortWidth "Port Dimensions [-]"; TimeStep "Upload Period [s]"
      mask help: Sends signal(s) from Simulink to the Sensor World
      mask Help:
      | Sends signal(s) from Simulink to the Sensor World.
      | 
      | - Port Name [-]: specifies the name of the output terminal of the Simulink block.
      | - Index [-]: specifies the start position in the output vector sent to the Sensor World
      | - Port dimensions [-]: specifies the width (number of scalars) of the output port
      | - Upload period [s]: specifies the upload period (in seconds) of the port.
      mask Display: port_label('input', 1, PortName)
  Velocity : Subsystem  mask(ToSensorWorld){PortName=Velocity_BMW_X5_1, PortIndex=3, PortWidth=3, TimeStep=1/60}
      mask prompts: PortName "Port Name [-]"; PortIndex "Index [-]"; PortWidth "Port Dimensions [-]"; TimeStep "Upload Period [s]"
      mask help: Sends signal(s) from Simulink to the Sensor World
      mask Help:
      | Sends signal(s) from Simulink to the Sensor World.
      | 
      | - Port Name [-]: specifies the name of the output terminal of the Simulink block.
      | - Index [-]: specifies the start position in the output vector sent to the Sensor World
      | - Port dimensions [-]: specifies the width (number of scalars) of the output port
      | - Upload period [s]: specifies the upload period (in seconds) of the port.
      mask Display: port_label('input', 1, PortName)
  iniBODYAngles wrtVEH [rad] : Constant  Value=[Roll0 Pitch0 0]  SampleTime=TimeStep
  iniVEHAngles wrtGLOB [rad] : Constant  Value=[0 0 Yaw0]  SampleTime=TimeStep
  iniVEHposition wrtGLOB [m] : Constant  Value=[x0 y0 z0]  SampleTime=TimeStep
  state2FullState : PreScanSimulinkLibrary/state2FullState  SystemSampleTime=-1
  velRPY : Subsystem  mask(ToSensorWorld){PortName=velRPY_BMW_X5_1, PortIndex=12, PortWidth=3, TimeStep=1/60}
      mask prompts: PortName "Port Name [-]"; PortIndex "Index [-]"; PortWidth "Port Dimensions [-]"; TimeStep "Upload Period [s]"
      mask help: Sends signal(s) from Simulink to the Sensor World
      mask Help:
      | Sends signal(s) from Simulink to the Sensor World.
      | 
      | - Port Name [-]: specifies the name of the output terminal of the Simulink block.
      | - Index [-]: specifies the start position in the output vector sent to the Sensor World
      | - Port dimensions [-]: specifies the width (number of scalars) of the output port
      | - Upload period [s]: specifies the upload period (in seconds) of the port.
      mask Display: port_label('input', 1, PortName)
  wires:
  Demux/5 -> velRPY/1(Y)
  Demux/4 -> RPY/1(Y)
  Demux/3 -> Acceleration/1(Y)
  Demux/2 -> Velocity/1(Y)
  Demux/1 -> Position/1(Y)
  State/1 -> state2FullState/1
  state2FullState/1 -> Demux/1
  iniVEHposition wrtGLOB [m]/1 -> state2FullState/2
  iniBODYAngles wrtVEH [rad]/1 -> state2FullState/3
  iniVEHAngles wrtGLOB [rad]/1 -> state2FullState/4

== system Demo_TA2_cs/STATE_Box_1 ==
  State : Inport  SampleTime=TimeStep
  Acceleration : Subsystem  mask(ToSensorWorld){PortName=Acceleration_Box_1, PortIndex=21, PortWidth=3, TimeStep=1/60}
      mask prompts: PortName "Port Name [-]"; PortIndex "Index [-]"; PortWidth "Port Dimensions [-]"; TimeStep "Upload Period [s]"
      mask help: Sends signal(s) from Simulink to the Sensor World
      mask Help:
      | Sends signal(s) from Simulink to the Sensor World.
      | 
      | - Port Name [-]: specifies the name of the output terminal of the Simulink block.
      | - Index [-]: specifies the start position in the output vector sent to the Sensor World
      | - Port dimensions [-]: specifies the width (number of scalars) of the output port
      | - Upload period [s]: specifies the upload period (in seconds) of the port.
      mask Display: port_label('input', 1, PortName)
  Demux : Demux  Outputs=5
  Position : Subsystem  mask(ToSensorWorld){PortName=Position_Box_1, PortIndex=15, PortWidth=3, TimeStep=1/60}
      mask prompts: PortName "Port Name [-]"; PortIndex "Index [-]"; PortWidth "Port Dimensions [-]"; TimeStep "Upload Period [s]"
      mask help: Sends signal(s) from Simulink to the Sensor World
      mask Help:
      | Sends signal(s) from Simulink to the Sensor World.
      | 
      | - Port Name [-]: specifies the name of the output terminal of the Simulink block.
      | - Index [-]: specifies the start position in the output vector sent to the Sensor World
      | - Port dimensions [-]: specifies the width (number of scalars) of the output port
      | - Upload period [s]: specifies the upload period (in seconds) of the port.
      mask Display: port_label('input', 1, PortName)
  RPY : Subsystem  mask(ToSensorWorld){PortName=RPY_Box_1, PortIndex=24, PortWidth=3, TimeStep=1/60}
      mask prompts: PortName "Port Name [-]"; PortIndex "Index [-]"; PortWidth "Port Dimensions [-]"; TimeStep "Upload Period [s]"
      mask help: Sends signal(s) from Simulink to the Sensor World
      mask Help:
      | Sends signal(s) from Simulink to the Sensor World.
      | 
      | - Port Name [-]: specifies the name of the output terminal of the Simulink block.
      | - Index [-]: specifies the start position in the output vector sent to the Sensor World
      | - Port dimensions [-]: specifies the width (number of scalars) of the output port
      | - Upload period [s]: specifies the upload period (in seconds) of the port.
      mask Display: port_label('input', 1, PortName)
  Velocity : Subsystem  mask(ToSensorWorld){PortName=Velocity_Box_1, PortIndex=18, PortWidth=3, TimeStep=1/60}
      mask prompts: PortName "Port Name [-]"; PortIndex "Index [-]"; PortWidth "Port Dimensions [-]"; TimeStep "Upload Period [s]"
      mask help: Sends signal(s) from Simulink to the Sensor World
      mask Help:
      | Sends signal(s) from Simulink to the Sensor World.
      | 
      | - Port Name [-]: specifies the name of the output terminal of the Simulink block.
      | - Index [-]: specifies the start position in the output vector sent to the Sensor World
      | - Port dimensions [-]: specifies the width (number of scalars) of the output port
      | - Upload period [s]: specifies the upload period (in seconds) of the port.
      mask Display: port_label('input', 1, PortName)
  iniBODYAngles wrtVEH [rad] : Constant  Value=[Roll0 Pitch0 0]  SampleTime=TimeStep
  iniVEHAngles wrtGLOB [rad] : Constant  Value=[0 0 Yaw0]  SampleTime=TimeStep
  iniVEHposition wrtGLOB [m] : Constant  Value=[x0 y0 z0]  SampleTime=TimeStep
  state2FullState : PreScanSimulinkLibrary/state2FullState  SystemSampleTime=-1
  velRPY : Subsystem  mask(ToSensorWorld){PortName=velRPY_Box_1, PortIndex=27, PortWidth=3, TimeStep=1/60}
      mask prompts: PortName "Port Name [-]"; PortIndex "Index [-]"; PortWidth "Port Dimensions [-]"; TimeStep "Upload Period [s]"
      mask help: Sends signal(s) from Simulink to the Sensor World
      mask Help:
      | Sends signal(s) from Simulink to the Sensor World.
      | 
      | - Port Name [-]: specifies the name of the output terminal of the Simulink block.
      | - Index [-]: specifies the start position in the output vector sent to the Sensor World
      | - Port dimensions [-]: specifies the width (number of scalars) of the output port
      | - Upload period [s]: specifies the upload period (in seconds) of the port.
      mask Display: port_label('input', 1, PortName)
  wires:
  Demux/5 -> velRPY/1(Y)
  Demux/4 -> RPY/1(Y)
  Demux/3 -> Acceleration/1(Y)
  Demux/2 -> Velocity/1(Y)
  Demux/1 -> Position/1(Y)
  State/1 -> state2FullState/1
  state2FullState/1 -> Demux/1
  iniVEHposition wrtGLOB [m]/1 -> state2FullState/2
  iniBODYAngles wrtVEH [rad]/1 -> state2FullState/3
  iniVEHAngles wrtGLOB [rad]/1 -> state2FullState/4

== system Demo_TA2_cs/SetActuators ==
  Bus Creator : BusCreator  Inputs=1
  Data Store Read : DataStoreRead  DataStoreName=SimCoreActuators  SampleTime=TimeStep
  SendActuators : M-S-Function  FunctionName=SendActuatorsBlock  Parameters=TimeStep NrOfActuators
  dummy : Outport
  tag scope: SimCoreInfo=global
  wires:
  Bus Creator/1 -> [SimCoreInfo]  "SimCore"
  SendActuators/2 -> Bus Creator/1  "ComputationTime[s]"
  SendActuators/1 -> dummy/1
  Data Store Read/1 -> SendActuators/1

== system Demo_TA2_cs/SimCoreInfo ==
  Bus Selector : BusSelector  OutputSignals=ComputationTime[s]
  Time : Scope
      settings: TimeRange=10  YMin=0  YMax=0.5  SaveName=ComputationTime
  wires:
  Bus Selector/1 -> Time/1  "<ComputationTime[s]>"
  [SimCoreInfo] -> Bus Selector/1

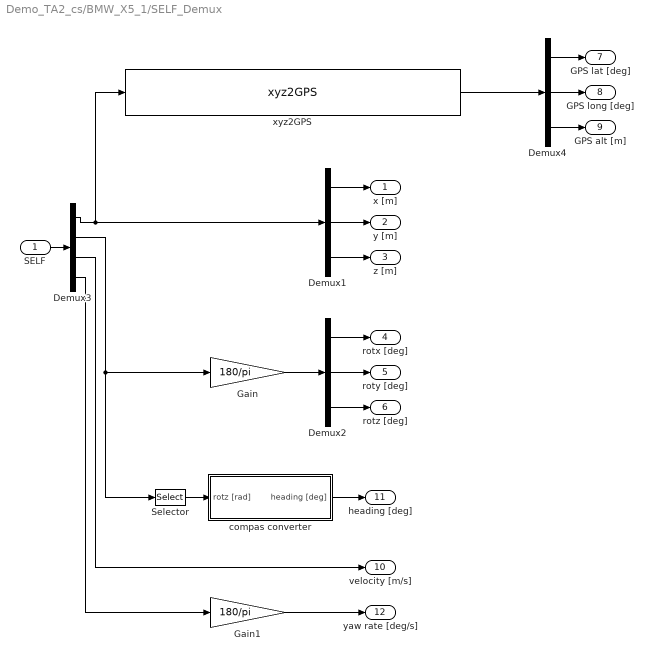
== system Demo_TA2_cs/BMW_X5_1/SELF_Demux ==
  SELF : Inport
  Demux1 : Demux  Outputs=3
  Demux2 : Demux  Outputs=3
  Demux3 : Demux  Outputs=[3 3 1 1]
  Demux4 : Demux  Outputs=3
  Gain : Gain  Gain=180/pi
  Gain1 : Gain  Gain=180/pi
  Selector : Selector  InputPortWidth=3  IndexOptions=Index vector (dialog)  Indices=[3]  OutputSizes=1
  compas converter : Subsystem
  xyz2GPS : PreScanUsefulBlocks/xyz2GPS  CoordinateCount=1  GPS_base=[0.000000 0.000000 0.000]
  x [m] : Outport
  y [m] : Outport  Port=2
  z [m] : Outport  Port=3
  rotx [deg] : Outport  Port=4
  roty [deg] : Outport  Port=5
  rotz [deg] : Outport  Port=6
  GPS lat [deg] : Outport  Port=7
  GPS long [deg] : Outport  Port=8
  GPS alt [m] : Outport  Port=9
  velocity [m/s] : Outport  Port=10
  heading [deg] : Outport  Port=11
  yaw rate [deg/s] : Outport  Port=12
  wires:
  Demux3/4 -> Gain1/1
  Gain1/1 -> yaw rate [deg/s]/1
  Demux3/3 -> velocity [m/s]/1
  compas converter/1(heading [deg]) -> heading [deg]/1
  xyz2GPS/1 -> Demux4/1
  Demux4/3 -> GPS alt [m]/1
  Demux4/2 -> GPS long [deg]/1
  Demux4/1 -> GPS lat [deg]/1
  Demux3/2 -> Gain/1, Selector/1
  Demux3/1 -> xyz2GPS/1, Demux1/1
  SELF/1 -> Demux3/1
  Demux2/3 -> rotz [deg]/1
  Demux2/2 -> roty [deg]/1
  Demux2/1 -> rotx [deg]/1
  Demux1/3 -> z [m]/1
  Demux1/2 -> y [m]/1
  Demux1/1 -> x [m]/1
  Gain/1 -> Demux2/1
  Selector/1 -> compas converter/1(rotz [rad])

== system Demo_TA2_cs/BMW_X5_1/TIS_1_Standard_Demux ==
  Radar : Inport
  Bus Creator : BusCreator  Inputs=6
  Bus Selector : BusSelector  OutputSignals=ActiveBeamID[-],Range[m],Theta[deg],Phi[deg],TargetID[-],TargetTypeID[-]
  ScannerSensorLegacyBusConversion : PreScanUsefulBlocks/ScannerSensorLegacyBusConversion  SystemSampleTime=-1  MAXMESSAGES=MAXMESSAGES
  Out1 : Outport
  Out2 : Outport  Port=2
  Out3 : Outport  Port=3
  Out4 : Outport  Port=4
  Out5 : Outport  Port=5
  Out6 : Outport  Port=6
  wires:
  Bus Selector/2 -> Bus Creator/2, Out2/1  "<Range[m]>"
  Bus Selector/1 -> Bus Creator/1, Out1/1  "<ActiveBeamID[-]>"
  ScannerSensorLegacyBusConversion/1 -> Bus Selector/1
  Radar/1 -> ScannerSensorLegacyBusConversion/1
  Bus Selector/6 -> Bus Creator/6  "<TargetTypeID[-]>"
  Bus Creator/1 -> Out6/1
  Bus Selector/5 -> Bus Creator/5, Out5/1  "<TargetID[-]>"
  Bus Selector/4 -> Out4/1, Bus Creator/4  "<Phi[deg]>"
  Bus Selector/3 -> Out3/1, Bus Creator/3  "<Theta[deg]>"

== system Demo_TA2_cs/BMW_X5_1/Trajectories ==
  SelectTraj : Constant  Tag=TrajSelector
  Switch : MultiPortSwitch  Tag=TrajSwitch  Inputs=2  zeroidx=off
  Traj2State1 : Subsystem  Tag=Traj2State
      settings: DeleteFcn=PreScanBlockDeleteFcn;
      mask Type: PreScan Demux Block:
  Traj2State2 : Subsystem  Tag=Traj2State
      settings: DeleteFcn=PreScanBlockDeleteFcn;
      mask Type: PreScan Demux Block:
  Trajectory_1 : Subsystem  Tag=Trajectory  mask(PreScan Source Block: Trajectory){FileName='Trajectory_1.mat', TimeStep=1/60}
      mask prompts: TimeStep "Time Step [s]"
      mask help:
      | The Trajectory block contains the trajectories defined in the PreScan Experiment Editor. The output of the trajectory block is the (vehicle) State.
      |
      | For more information, please click Help.
      mask init:
      | [direc,name]=fileparts(get_param(bdroot, 'FileName'));
      | load([direc,'/Trajectories/',FileName])
      | trajectory=trajectory';
      | 
      | traj.time=trajectory(:,1);%[];
      | traj.signals.values=trajectory(:,2:19);
      | traj.dimensions=18;
      | traj.label='';
      | 
      | SampleTime=traj.time(2)-traj.time(1);
      settings: DeleteFcn=PreScanBlockDeleteFcn;
      mask Help: eval('openHelp(312)')
      mask Display: fprintf(FileName)
  Trajectory_1_Offset : Constant  Tag=TrajectoryOffset  Value="[0  0  0  0  0  0]"
  Trajectory_2 : Subsystem  Tag=Trajectory  mask(PreScan Source Block: Trajectory){FileName='Trajectory_2.mat', TimeStep=1/60}
      mask prompts: TimeStep "Time Step [s]"
      mask help:
      | The Trajectory block contains the trajectories defined in the PreScan Experiment Editor. The output of the trajectory block is the (vehicle) State.
      |
      | For more information, please click Help.
      mask init: same as Demo_TA2_cs/BMW_X5_1/Trajectories/Trajectory_1
      settings: DeleteFcn=PreScanBlockDeleteFcn;
      mask Help: eval('openHelp(312)')
      mask Display: fprintf(FileName)
  Trajectory_2_Offset : Constant  Tag=TrajectoryOffset  Value="[0  0  0  0  0  0]"
  State : Outport  Tag=TrajOutport
  wires:
  Trajectory_1/1(trajectory) -> Traj2State1/1(Traj Org)
  Trajectory_1_Offset/1 -> Traj2State1/2(Offset)
  Traj2State1/1(state) -> Switch/2
  Trajectory_2/1(trajectory) -> Traj2State2/1(Traj Org)
  Trajectory_2_Offset/1 -> Traj2State2/2(Offset)
  Traj2State2/1(state) -> Switch/3
  SelectTraj/1 -> Switch/1
  Switch/1 -> State/1

== system Demo_TA2_cs/Box_1/Dynamics_Empty ==
  note: For state mode 'Dynamic' positions
      | are not taken into account, as they
      | are computed by integrating velocity.
      | Click annotation for Help.
  Ground_{1..9} (9 alike) : Ground
  MuxState : Subsystem  Tag=MuxState  mask{positioningmode=off, TimeStep=1/60}
      mask prompts: positioningmode "Positioning Mode"; TimeStep "Auto Assigned: Time Step [s]"
      settings: DeleteFcn=PreScanBlockDeleteFcn;
  State : Outport  Tag=StateOutport
  wires:
  MuxState/1(state) -> State/1
  Ground_1/1 -> MuxState/1(x [m])
  Ground_2/1 -> MuxState/2(y [m])
  Ground_3/1 -> MuxState/3(z [m])
  Ground_4/1 -> MuxState/4(dx [m/s])
  Ground_5/1 -> MuxState/5(dy [m/s])
  Ground_6/1 -> MuxState/6(dz [m/s])
  Ground_7/1 -> MuxState/7(R [rad])
  Ground_8/1 -> MuxState/8(P [rad])
  Ground_9/1 -> MuxState/9(Y [rad])

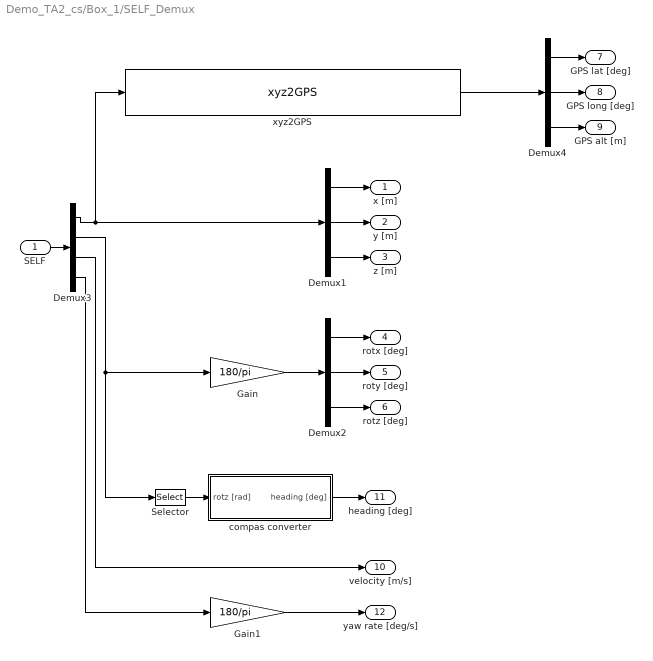
== system Demo_TA2_cs/Box_1/SELF_Demux ==
  SELF : Inport
  Demux1 : Demux  Outputs=3
  Demux2 : Demux  Outputs=3
  Demux3 : Demux  Outputs=[3 3 1 1]
  Demux4 : Demux  Outputs=3
  Gain : Gain  Gain=180/pi
  Gain1 : Gain  Gain=180/pi
  Selector : Selector  InputPortWidth=3  IndexOptions=Index vector (dialog)  Indices=[3]  OutputSizes=1
  compas converter : Subsystem
  xyz2GPS : PreScanUsefulBlocks/xyz2GPS  CoordinateCount=1  GPS_base=[0.000000 0.000000 0.000]
  x [m] : Outport
  y [m] : Outport  Port=2
  z [m] : Outport  Port=3
  rotx [deg] : Outport  Port=4
  roty [deg] : Outport  Port=5
  rotz [deg] : Outport  Port=6
  GPS lat [deg] : Outport  Port=7
  GPS long [deg] : Outport  Port=8
  GPS alt [m] : Outport  Port=9
  velocity [m/s] : Outport  Port=10
  heading [deg] : Outport  Port=11
  yaw rate [deg/s] : Outport  Port=12
  wires:
  Demux3/4 -> Gain1/1
  Gain1/1 -> yaw rate [deg/s]/1
  Demux3/3 -> velocity [m/s]/1
  compas converter/1(heading [deg]) -> heading [deg]/1
  xyz2GPS/1 -> Demux4/1
  Demux4/3 -> GPS alt [m]/1
  Demux4/2 -> GPS long [deg]/1
  Demux4/1 -> GPS lat [deg]/1
  Demux3/2 -> Gain/1, Selector/1
  Demux3/1 -> xyz2GPS/1, Demux1/1
  SELF/1 -> Demux3/1
  Demux2/3 -> rotz [deg]/1
  Demux2/2 -> roty [deg]/1
  Demux2/1 -> rotx [deg]/1
  Demux1/3 -> z [m]/1
  Demux1/2 -> y [m]/1
  Demux1/1 -> x [m]/1
  Gain/1 -> Demux2/1
  Selector/1 -> compas converter/1(rotz [rad])

== system Demo_TA2_cs/STATE_BMW_X5_1/Acceleration ==
  Y : Inport
  Assignment : Assignment  IndexMode=Zero-based  SampleTime=TimeStep  IndexOptions=Starting index (dialog)  Indices=PortIndex  OutputSizes=[1 1]
  Data Store Read : DataStoreRead  DataStoreName=SimCoreActuators  SampleTime=TimeStep
  Data Store Write : DataStoreWrite  DataStoreName=SimCoreActuators
  wires:
  Assignment/1 -> Data Store Write/1
  Data Store Read/1 -> Assignment/1
  Y/1 -> Assignment/2

== system Demo_TA2_cs/STATE_BMW_X5_1/Position ==
  Y : Inport
  Assignment : Assignment  IndexMode=Zero-based  SampleTime=TimeStep  IndexOptions=Starting index (dialog)  Indices=PortIndex  OutputSizes=[1 1]
  Data Store Read : DataStoreRead  DataStoreName=SimCoreActuators  SampleTime=TimeStep
  Data Store Write : DataStoreWrite  DataStoreName=SimCoreActuators
  wires:
  Y/1 -> Assignment/2
  Data Store Read/1 -> Assignment/1
  Assignment/1 -> Data Store Write/1

== system Demo_TA2_cs/STATE_BMW_X5_1/RPY ==
  Y : Inport
  Assignment : Assignment  IndexMode=Zero-based  SampleTime=TimeStep  IndexOptions=Starting index (dialog)  Indices=PortIndex  OutputSizes=[1 1]
  Data Store Read : DataStoreRead  DataStoreName=SimCoreActuators  SampleTime=TimeStep
  Data Store Write : DataStoreWrite  DataStoreName=SimCoreActuators
  wires:
  Assignment/1 -> Data Store Write/1
  Data Store Read/1 -> Assignment/1
  Y/1 -> Assignment/2

== system Demo_TA2_cs/STATE_BMW_X5_1/Velocity ==
  Y : Inport
  Assignment : Assignment  IndexMode=Zero-based  SampleTime=TimeStep  IndexOptions=Starting index (dialog)  Indices=PortIndex  OutputSizes=[1 1]
  Data Store Read : DataStoreRead  DataStoreName=SimCoreActuators  SampleTime=TimeStep
  Data Store Write : DataStoreWrite  DataStoreName=SimCoreActuators
  wires:
  Assignment/1 -> Data Store Write/1
  Data Store Read/1 -> Assignment/1
  Y/1 -> Assignment/2

== system Demo_TA2_cs/STATE_BMW_X5_1/velRPY ==
  Y : Inport
  Assignment : Assignment  IndexMode=Zero-based  SampleTime=TimeStep  IndexOptions=Starting index (dialog)  Indices=PortIndex  OutputSizes=[1 1]
  Data Store Read : DataStoreRead  DataStoreName=SimCoreActuators  SampleTime=TimeStep
  Data Store Write : DataStoreWrite  DataStoreName=SimCoreActuators
  wires:
  Assignment/1 -> Data Store Write/1
  Data Store Read/1 -> Assignment/1
  Y/1 -> Assignment/2

== system Demo_TA2_cs/STATE_Box_1/Acceleration ==
  Y : Inport
  Assignment : Assignment  IndexMode=Zero-based  SampleTime=TimeStep  IndexOptions=Starting index (dialog)  Indices=PortIndex  OutputSizes=[1 1]
  Data Store Read : DataStoreRead  DataStoreName=SimCoreActuators  SampleTime=TimeStep
  Data Store Write : DataStoreWrite  DataStoreName=SimCoreActuators
  wires:
  Assignment/1 -> Data Store Write/1
  Data Store Read/1 -> Assignment/1
  Y/1 -> Assignment/2

== system Demo_TA2_cs/STATE_Box_1/Position ==
  Y : Inport
  Assignment : Assignment  IndexMode=Zero-based  SampleTime=TimeStep  IndexOptions=Starting index (dialog)  Indices=PortIndex  OutputSizes=[1 1]
  Data Store Read : DataStoreRead  DataStoreName=SimCoreActuators  SampleTime=TimeStep
  Data Store Write : DataStoreWrite  DataStoreName=SimCoreActuators
  wires:
  Y/1 -> Assignment/2
  Data Store Read/1 -> Assignment/1
  Assignment/1 -> Data Store Write/1

== system Demo_TA2_cs/STATE_Box_1/RPY ==
  Y : Inport
  Assignment : Assignment  IndexMode=Zero-based  SampleTime=TimeStep  IndexOptions=Starting index (dialog)  Indices=PortIndex  OutputSizes=[1 1]
  Data Store Read : DataStoreRead  DataStoreName=SimCoreActuators  SampleTime=TimeStep
  Data Store Write : DataStoreWrite  DataStoreName=SimCoreActuators
  wires:
  Assignment/1 -> Data Store Write/1
  Data Store Read/1 -> Assignment/1
  Y/1 -> Assignment/2

== system Demo_TA2_cs/STATE_Box_1/Velocity ==
  Y : Inport
  Assignment : Assignment  IndexMode=Zero-based  SampleTime=TimeStep  IndexOptions=Starting index (dialog)  Indices=PortIndex  OutputSizes=[1 1]
  Data Store Read : DataStoreRead  DataStoreName=SimCoreActuators  SampleTime=TimeStep
  Data Store Write : DataStoreWrite  DataStoreName=SimCoreActuators
  wires:
  Assignment/1 -> Data Store Write/1
  Data Store Read/1 -> Assignment/1
  Y/1 -> Assignment/2

== system Demo_TA2_cs/STATE_Box_1/velRPY ==
  Y : Inport
  Assignment : Assignment  IndexMode=Zero-based  SampleTime=TimeStep  IndexOptions=Starting index (dialog)  Indices=PortIndex  OutputSizes=[1 1]
  Data Store Read : DataStoreRead  DataStoreName=SimCoreActuators  SampleTime=TimeStep
  Data Store Write : DataStoreWrite  DataStoreName=SimCoreActuators
  wires:
  Assignment/1 -> Data Store Write/1
  Data Store Read/1 -> Assignment/1
  Y/1 -> Assignment/2

== system Demo_TA2_cs/BMW_X5_1/SELF_Demux/compas converter ==
  rotz [rad] : Inport
  cart2compas : Subsystem
  rad2deg : Gain  Gain=180/pi
  heading [deg] : Outport
  wires:
  cart2compas/1(heading [deg]) -> heading [deg]/1
  rotz [rad]/1 -> rad2deg/1
  rad2deg/1 -> cart2compas/1(Angle [deg])

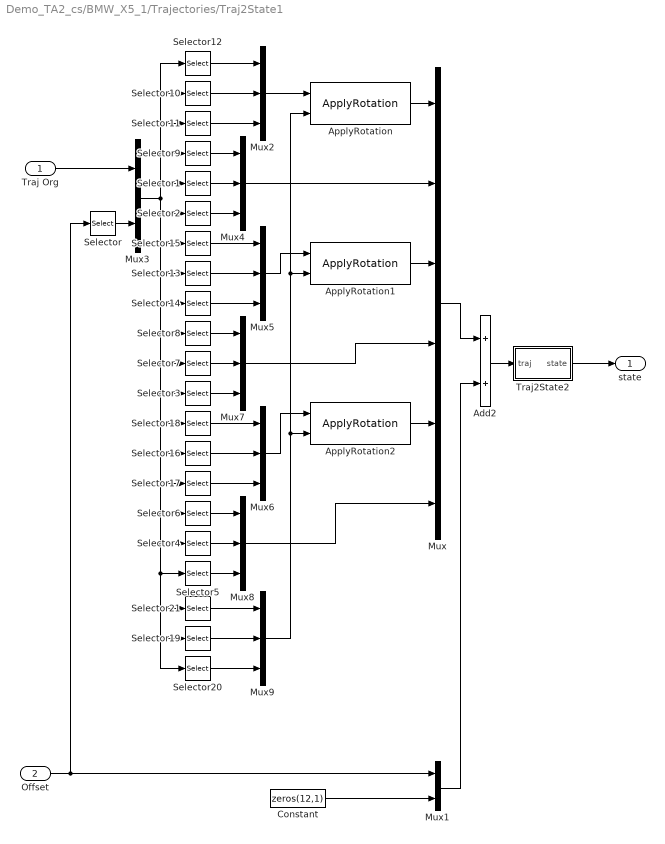
== system Demo_TA2_cs/BMW_X5_1/Trajectories/Traj2State1 ==
  Traj Org : Inport
  Offset : Inport  Port=2
  Add2 : Sum
  ApplyRotation : PreScanSimulinkLibrary/ApplyRotation  SystemSampleTime=-1
  ApplyRotation1 : PreScanSimulinkLibrary/ApplyRotation  SystemSampleTime=-1
  ApplyRotation2 : PreScanSimulinkLibrary/ApplyRotation  SystemSampleTime=-1
  Constant : Constant  Value=zeros(12,1)
  Mux : Mux  Inputs=6
  Mux1 : Mux  Inputs=2
  Mux{2,4..9} (7 alike) : Mux  Inputs=3
  Mux3 : Mux  Inputs=2
  Selector : Selector  InputPortWidth=6  IndexOptions=Index vector (dialog)  Indices=[4 5 6]  OutputSizes=1
  Selector1 : Selector  InputPortWidth=21  IndexOptions=Index vector (dialog)  Indices=[5]  OutputSizes=1
  Selector10 : Selector  InputPortWidth=21  IndexOptions=Index vector (dialog)  Indices=[2]  OutputSizes=1
  Selector11 : Selector  InputPortWidth=21  IndexOptions=Index vector (dialog)  Indices=[3]  OutputSizes=1
  Selector12 : Selector  InputPortWidth=21  IndexOptions=Index vector (dialog)  Indices=[1]  OutputSizes=1
  Selector13 : Selector  InputPortWidth=21  IndexOptions=Index vector (dialog)  Indices=[8]  OutputSizes=1
  Selector14 : Selector  InputPortWidth=21  IndexOptions=Index vector (dialog)  Indices=[9]  OutputSizes=1
  Selector15 : Selector  InputPortWidth=21  IndexOptions=Index vector (dialog)  Indices=[7]  OutputSizes=1
  Selector16 : Selector  InputPortWidth=21  IndexOptions=Index vector (dialog)  Indices=[14]  OutputSizes=1
  Selector17 : Selector  InputPortWidth=21  IndexOptions=Index vector (dialog)  Indices=[15]  OutputSizes=1
  Selector18 : Selector  InputPortWidth=21  IndexOptions=Index vector (dialog)  Indices=[13]  OutputSizes=1
  Selector19 : Selector  InputPortWidth=21  IndexOptions=Index vector (dialog)  Indices=[20]  OutputSizes=1
  Selector2 : Selector  InputPortWidth=21  IndexOptions=Index vector (dialog)  Indices=[6]  OutputSizes=1
  Selector20 : Selector  InputPortWidth=21  IndexOptions=Index vector (dialog)  Indices=[21]  OutputSizes=1
  Selector21 : Selector  InputPortWidth=21  IndexOptions=Index vector (dialog)  Indices=[19]  OutputSizes=1
  Selector3 : Selector  InputPortWidth=21  IndexOptions=Index vector (dialog)  Indices=[12]  OutputSizes=1
  Selector4 : Selector  InputPortWidth=21  IndexOptions=Index vector (dialog)  Indices=[17]  OutputSizes=1
  Selector5 : Selector  InputPortWidth=21  IndexOptions=Index vector (dialog)  Indices=[18]  OutputSizes=1
  Selector6 : Selector  InputPortWidth=21  IndexOptions=Index vector (dialog)  Indices=[16]  OutputSizes=1
  Selector7 : Selector  InputPortWidth=21  IndexOptions=Index vector (dialog)  Indices=[11]  OutputSizes=1
  Selector8 : Selector  InputPortWidth=21  IndexOptions=Index vector (dialog)  Indices=[10]  OutputSizes=1
  Selector9 : Selector  InputPortWidth=21  IndexOptions=Index vector (dialog)  Indices=[4]  OutputSizes=1
  Traj2State2 : Subsystem
  state : Outport
  wires:
  Mux9/1 -> ApplyRotation2/2, ApplyRotation1/2, ApplyRotation/2
  Selector20/1 -> Mux9/3
  Selector19/1 -> Mux9/2
  Selector21/1 -> Mux9/1
  Selector5/1 -> Mux8/3
  Selector4/1 -> Mux8/2
  Selector6/1 -> Mux8/1
  Mux8/1 -> Mux/6
  Mux6/1 -> ApplyRotation2/1
  Mux7/1 -> Mux/4
  ApplyRotation2/1 -> Mux/5
  Selector3/1 -> Mux7/3
  Selector7/1 -> Mux7/2
  Selector8/1 -> Mux7/1
  Mux4/1 -> Mux/2
  Mux5/1 -> ApplyRotation1/1
  ApplyRotation1/1 -> Mux/3
  Mux2/1 -> ApplyRotation/1
  ApplyRotation/1 -> Mux/1
  Selector2/1 -> Mux4/3
  Selector1/1 -> Mux4/2
  Selector9/1 -> Mux4/1
  Selector17/1 -> Mux6/3
  Selector16/1 -> Mux6/2
  Selector18/1 -> Mux6/1
  Selector14/1 -> Mux5/3
  Selector13/1 -> Mux5/2
  Selector15/1 -> Mux5/1
  Selector11/1 -> Mux2/3
  Selector10/1 -> Mux2/2
  Selector12/1 -> Mux2/1
  Mux3/1 -> Selector8/1, Selector7/1, Selector3/1, Selector18/1, Selector16/1, Selector17/1, Selector6/1, Selector20/1, Selector19/1, Selector21/1, Selector5/1, Selector4/1, Selector14/1, Selector13/1, Selector15/1, Selector2/1, Selector1/1, Selector9/1, Selector12/1, Selector10/1, Selector11/1
  Mux1/1 -> Add2/2
  Constant/1 -> Mux1/2
  Add2/1 -> Traj2State2/1(traj)
  Selector/1 -> Mux3/2
  Traj Org/1 -> Mux3/1
  Offset/1 -> Mux1/1, Selector/1
  Mux/1 -> Add2/1
  Traj2State2/1(state) -> state/1

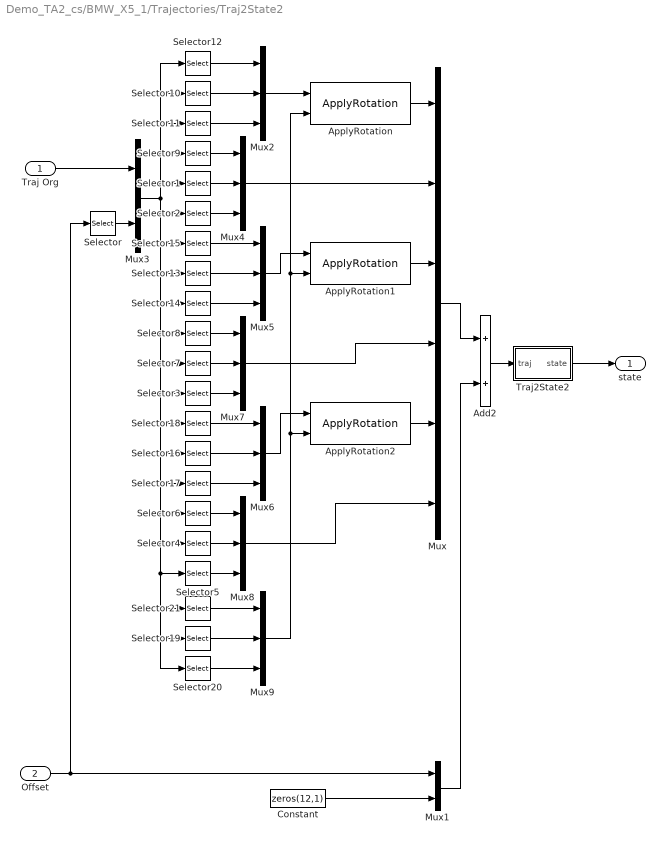
== system Demo_TA2_cs/BMW_X5_1/Trajectories/Traj2State2 ==
  Traj Org : Inport
  Offset : Inport  Port=2
  Add2 : Sum
  ApplyRotation : PreScanSimulinkLibrary/ApplyRotation  SystemSampleTime=-1
  ApplyRotation1 : PreScanSimulinkLibrary/ApplyRotation  SystemSampleTime=-1
  ApplyRotation2 : PreScanSimulinkLibrary/ApplyRotation  SystemSampleTime=-1
  Constant : Constant  Value=zeros(12,1)
  Mux : Mux  Inputs=6
  Mux1 : Mux  Inputs=2
  Mux{2,4..9} (7 alike) : Mux  Inputs=3
  Mux3 : Mux  Inputs=2
  Selector : Selector  InputPortWidth=6  IndexOptions=Index vector (dialog)  Indices=[4 5 6]  OutputSizes=1
  Selector1 : Selector  InputPortWidth=21  IndexOptions=Index vector (dialog)  Indices=[5]  OutputSizes=1
  Selector10 : Selector  InputPortWidth=21  IndexOptions=Index vector (dialog)  Indices=[2]  OutputSizes=1
  Selector11 : Selector  InputPortWidth=21  IndexOptions=Index vector (dialog)  Indices=[3]  OutputSizes=1
  Selector12 : Selector  InputPortWidth=21  IndexOptions=Index vector (dialog)  Indices=[1]  OutputSizes=1
  Selector13 : Selector  InputPortWidth=21  IndexOptions=Index vector (dialog)  Indices=[8]  OutputSizes=1
  Selector14 : Selector  InputPortWidth=21  IndexOptions=Index vector (dialog)  Indices=[9]  OutputSizes=1
  Selector15 : Selector  InputPortWidth=21  IndexOptions=Index vector (dialog)  Indices=[7]  OutputSizes=1
  Selector16 : Selector  InputPortWidth=21  IndexOptions=Index vector (dialog)  Indices=[14]  OutputSizes=1
  Selector17 : Selector  InputPortWidth=21  IndexOptions=Index vector (dialog)  Indices=[15]  OutputSizes=1
  Selector18 : Selector  InputPortWidth=21  IndexOptions=Index vector (dialog)  Indices=[13]  OutputSizes=1
  Selector19 : Selector  InputPortWidth=21  IndexOptions=Index vector (dialog)  Indices=[20]  OutputSizes=1
  Selector2 : Selector  InputPortWidth=21  IndexOptions=Index vector (dialog)  Indices=[6]  OutputSizes=1
  Selector20 : Selector  InputPortWidth=21  IndexOptions=Index vector (dialog)  Indices=[21]  OutputSizes=1
  Selector21 : Selector  InputPortWidth=21  IndexOptions=Index vector (dialog)  Indices=[19]  OutputSizes=1
  Selector3 : Selector  InputPortWidth=21  IndexOptions=Index vector (dialog)  Indices=[12]  OutputSizes=1
  Selector4 : Selector  InputPortWidth=21  IndexOptions=Index vector (dialog)  Indices=[17]  OutputSizes=1
  Selector5 : Selector  InputPortWidth=21  IndexOptions=Index vector (dialog)  Indices=[18]  OutputSizes=1
  Selector6 : Selector  InputPortWidth=21  IndexOptions=Index vector (dialog)  Indices=[16]  OutputSizes=1
  Selector7 : Selector  InputPortWidth=21  IndexOptions=Index vector (dialog)  Indices=[11]  OutputSizes=1
  Selector8 : Selector  InputPortWidth=21  IndexOptions=Index vector (dialog)  Indices=[10]  OutputSizes=1
  Selector9 : Selector  InputPortWidth=21  IndexOptions=Index vector (dialog)  Indices=[4]  OutputSizes=1
  Traj2State2 : Subsystem
  state : Outport
  wires:
  Mux9/1 -> ApplyRotation2/2, ApplyRotation1/2, ApplyRotation/2
  Selector20/1 -> Mux9/3
  Selector19/1 -> Mux9/2
  Selector21/1 -> Mux9/1
  Selector5/1 -> Mux8/3
  Selector4/1 -> Mux8/2
  Selector6/1 -> Mux8/1
  Mux8/1 -> Mux/6
  Mux6/1 -> ApplyRotation2/1
  Mux7/1 -> Mux/4
  ApplyRotation2/1 -> Mux/5
  Selector3/1 -> Mux7/3
  Selector7/1 -> Mux7/2
  Selector8/1 -> Mux7/1
  Mux4/1 -> Mux/2
  Mux5/1 -> ApplyRotation1/1
  ApplyRotation1/1 -> Mux/3
  Mux2/1 -> ApplyRotation/1
  ApplyRotation/1 -> Mux/1
  Selector2/1 -> Mux4/3
  Selector1/1 -> Mux4/2
  Selector9/1 -> Mux4/1
  Selector17/1 -> Mux6/3
  Selector16/1 -> Mux6/2
  Selector18/1 -> Mux6/1
  Selector14/1 -> Mux5/3
  Selector13/1 -> Mux5/2
  Selector15/1 -> Mux5/1
  Selector11/1 -> Mux2/3
  Selector10/1 -> Mux2/2
  Selector12/1 -> Mux2/1
  Mux3/1 -> Selector8/1, Selector7/1, Selector3/1, Selector18/1, Selector16/1, Selector17/1, Selector6/1, Selector20/1, Selector19/1, Selector21/1, Selector5/1, Selector4/1, Selector14/1, Selector13/1, Selector15/1, Selector2/1, Selector1/1, Selector9/1, Selector12/1, Selector10/1, Selector11/1
  Mux1/1 -> Add2/2
  Constant/1 -> Mux1/2
  Add2/1 -> Traj2State2/1(traj)
  Selector/1 -> Mux3/2
  Traj Org/1 -> Mux3/1
  Offset/1 -> Mux1/1, Selector/1
  Mux/1 -> Add2/1
  Traj2State2/1(state) -> state/1

== system Demo_TA2_cs/BMW_X5_1/Trajectories/Trajectory_1 ==
  From Workspace : FromWorkspace  VariableName=trajectory  SampleTime=TimeStep  OutputAfterFinalValue=Holding final value
  From Workspace1 : FromWorkspace  VariableName=trajectory  SampleTime=TimeStep  OutputAfterFinalValue=Setting to zero
  Mux : Mux  Inputs=2
  Selector1 : Selector  InputPortWidth=24  IndexOptions=Index vector (dialog)  Indices=[7:18]  OutputSizes=1
  Selector9 : Selector  InputPortWidth=24  IndexOptions=Index vector (dialog)  Indices=[1:6]  OutputSizes=1
  trajectory : Outport
  wires:
  Selector1/1 -> Mux/2
  Selector9/1 -> Mux/1
  Mux/1 -> trajectory/1
  From Workspace1/1 -> Selector1/1
  From Workspace/1 -> Selector9/1

== system Demo_TA2_cs/BMW_X5_1/Trajectories/Trajectory_2 ==
  From Workspace : FromWorkspace  VariableName=trajectory  SampleTime=TimeStep  OutputAfterFinalValue=Holding final value
  From Workspace1 : FromWorkspace  VariableName=trajectory  SampleTime=TimeStep  OutputAfterFinalValue=Setting to zero
  Mux : Mux  Inputs=2
  Selector1 : Selector  InputPortWidth=24  IndexOptions=Index vector (dialog)  Indices=[7:18]  OutputSizes=1
  Selector9 : Selector  InputPortWidth=24  IndexOptions=Index vector (dialog)  Indices=[1:6]  OutputSizes=1
  trajectory : Outport
  wires:
  Selector1/1 -> Mux/2
  Selector9/1 -> Mux/1
  Mux/1 -> trajectory/1
  From Workspace1/1 -> Selector1/1
  From Workspace/1 -> Selector9/1

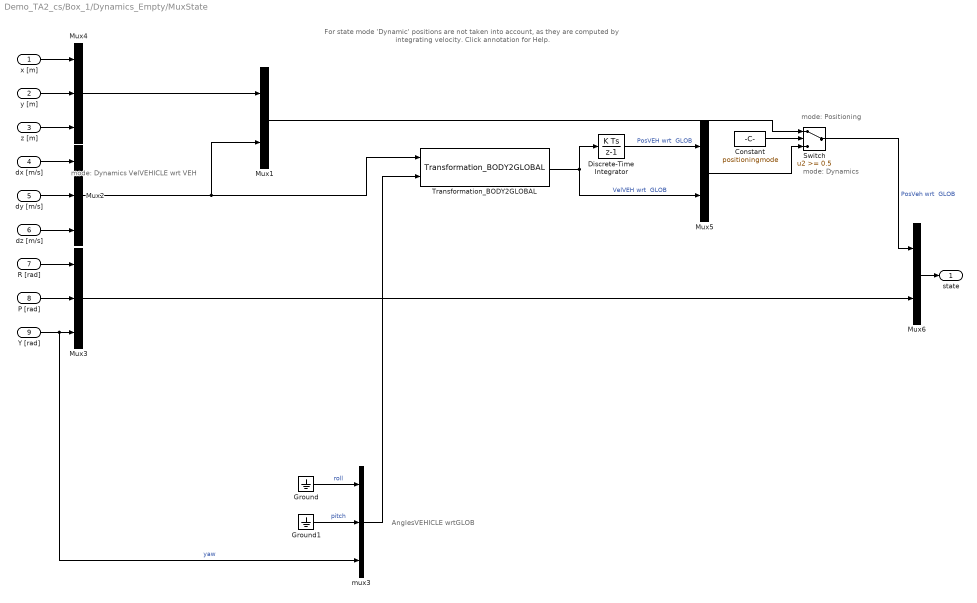
== system Demo_TA2_cs/Box_1/Dynamics_Empty/MuxState ==
  note: mode: Dynamics
  note: mode: Positioning
  note: mode: Dynamics
      | VelVEHICLE
      | wrt VEH
  note: AnglesVEHICLE
      | wrtGLOB
  note: For state mode 'Dynamic' positions
      | are not taken into account, as they
      | are computed by integrating velocity.
      | Click annotation for Help.
  x [m] : Inport  SampleTime=TimeStep
  y [m] : Inport  Port=2  SampleTime=TimeStep
  z [m] : Inport  Port=3  SampleTime=TimeStep
  dx [m/s] : Inport  Port=4  SampleTime=TimeStep
  dy [m/s] : Inport  Port=5  SampleTime=TimeStep
  dz [m/s] : Inport  Port=6  SampleTime=TimeStep
  R [rad] : Inport  Port=7  SampleTime=TimeStep
  P [rad] : Inport  Port=8  SampleTime=TimeStep
  Y [rad] : Inport  Port=9  SampleTime=TimeStep
  Constant : Constant  DisableCoverage=on  Value=positioningmode
  Discrete-Time Integrator : DiscreteIntegrator  SampleTime=TimeStep  ICPrevOutput=DiscIntNeverNeededParam  ICPrevScaledInput=DiscIntNeverNeededParam
  Ground : Ground
  Ground1 : Ground
  Mux1 : Mux  Inputs=[3 3]
  Mux2 : Mux  Inputs=3
  Mux3 : Mux  Inputs=3
  Mux4 : Mux  Inputs=3
  Mux5 : Mux  Inputs=[3 3]
  Mux6 : Mux  Inputs=[6 3]
  Switch : Switch  Threshold=0.5
  Transformation_BODY2GLOBAL : PreScanSimulinkLibrary/Simple_Vehicle_Dynamics/Chassis/MuxDynState/Transformation_BODY2GLOBAL  SystemSampleTime=-1
  mux3 : Mux  Inputs=3
  state : Outport
  wires:
  Constant/1 -> Switch/2
  Mux6/1 -> state/1
  Mux4/1 -> Mux1/1
  Mux5/1 -> Switch/3
  Mux1/1 -> Switch/1
  Switch/1 -> Mux6/1  "PosVeh wrt  GLOB"
  P [rad]/1 -> Mux3/2
  R [rad]/1 -> Mux3/1
  dz [m/s]/1 -> Mux2/3
  dy [m/s]/1 -> Mux2/2
  dx [m/s]/1 -> Mux2/1
  z [m]/1 -> Mux4/3
  y [m]/1 -> Mux4/2
  x [m]/1 -> Mux4/1
  Ground1/1 -> mux3/2  "pitch"
  Y [rad]/1 -> mux3/3, Mux3/3  "yaw"
  Mux3/1 -> Mux6/2
  Transformation_BODY2GLOBAL/1 -> Discrete-Time Integrator/1, Mux5/2  "VelVEH wrt  GLOB"
  mux3/1 -> Transformation_BODY2GLOBAL/2
  Ground/1 -> mux3/1  "roll"
  Mux2/1 -> Mux1/2, Transformation_BODY2GLOBAL/1
  Discrete-Time Integrator/1 -> Mux5/1  "PosVEH wrt  GLOB"

== system Demo_TA2_cs/Box_1/SELF_Demux/compas converter ==
  rotz [rad] : Inport
  cart2compas : Subsystem
  rad2deg : Gain  Gain=180/pi
  heading [deg] : Outport
  wires:
  cart2compas/1(heading [deg]) -> heading [deg]/1
  rotz [rad]/1 -> rad2deg/1
  rad2deg/1 -> cart2compas/1(Angle [deg])

== system Demo_TA2_cs/BMW_X5_1/SELF_Demux/compas converter/cart2compas ==
  Angle [deg] : Inport
  Constant : Constant  Value=90
  Constant1 : Constant  Value=360
  Gain : Gain  Gain=1/360
  Gain1 : Gain  Gain=360
  Gain2 : Gain  Gain=-1
  Rounding Function : Rounding
  Sum : Sum  Inputs=|-+
  Sum1 : Sum  Inputs=-+|
  Sum2 : Sum  Inputs=++|
  heading [deg] : Outport
  wires:
  Sum2/1 -> heading [deg]/1
  Constant1/1 -> Sum2/1
  Gain2/1 -> Sum2/2
  Constant/1 -> Sum1/1
  Sum1/1 -> Sum/2, Gain/1
  Sum/1 -> Gain2/1
  Angle [deg]/1 -> Sum1/2
  Gain1/1 -> Sum/1
  Rounding Function/1 -> Gain1/1
  Gain/1 -> Rounding Function/1
